simulink model "Board2_supervision"  (R2025b)
settings: Solver=FixedStepDiscrete  StartTime=0.0  StopTime=2  FixedStep=0.001  RelTol=1e-3
(part 2 of 2)

== stateflow chart Board2_supervision/Board2 ==
  state Supervision_task
    state Board_state [parallel]
      settings: executionOrder=1
      state Normal
        ex: Close_Session(); Lower_MTalk(); Abort_Communication();
        state Supervisor [parallel]
          settings: executionOrder=1
          state Waiting_comunication
            en: Update_Local_State(); Open_Session(); Raise_MTalk();
            time_comm = Get_Timestamp();
          state Transmit_Local_State
            en: Send_Local_State(); time_comm = Get_Timestamp();
          state Local_state_transmitted
            en: time_comm = Get_Timestamp();
          state Receive_state
            en: Wait_State(); Lower_MTalk(); time_comm = Get_Timestamp();
          state State_received
            en: Raise_MTalk(); time_comm = Get_Timestamp();
          state Transmit_Global_State
            en: Send_Global_State(); time_comm = Get_Timestamp();
          state Global_Local_state_transmitted
            en: time_comm = Get_Timestamp();
          state Receive_global_state
            en: Wait_Global_State(); Lower_MTalk(); time_comm = Get_Timestamp();
          state Same_decision
            en: Write_Output();
          state Global_state_received
            en: time_comm = Get_Timestamp();
          state Transmit_Decision
            en: Send_Decision(); time_comm = Get_Timestamp();
          state Decision_transmitted
            en: time_comm = Get_Timestamp();
          state Receive_decision
            en: Wait_Decision(); Lower_MTalk(); time_comm = Get_Timestamp();
          (default) -> Waiting_comunication
          (junction 6516) -> Waiting_comunication
          Waiting_comunication -> (junction 6517) [order 2] : [Check_Timeout_Us(time_comm, INITIAL_TIMEOUT)]
          Same_decision -> (junction 6516)
          (junction 6517) -> (junction 6543)
          Waiting_comunication -> Transmit_Local_State [order 1] : [~Is_STalk_High()]
              | {retransmitted = 0;}
          (junction 6556) -> Transmit_Local_State
          Transmit_Local_State -> (junction 6595) [order 2] : [Check_Timeout_Us(time_comm, STATE_SEND_TIMEOUT)]
          (junction 6595) -> (junction 6596)
          (junction 6554) -> (junction 6556) [order 1] : [retransmitted < MAX_RETRANSMIT]{retransmitted = retransmitted + 1;}
          Transmit_Local_State -> Local_state_transmitted [order 1] : [Is_Tx_Finished()]
          (junction 6554) -> (junction 6543) [order 2]
          Local_state_transmitted -> (junction 6554) [order 2] : [Check_Timeout_Us(time_comm, WAIT_TIMEOUT)]
          (junction 6543) -> (junction 6547)
          Local_state_transmitted -> Receive_state [order 1] : [Is_STalk_High()]
          (junction 6567) -> Receive_state
          Receive_state -> (junction 6547) [order 2] : [Check_Timeout_Us(time_comm, STATE_RECEIVE_TIMEOUT)]
          (junction 6566) -> (junction 6567)
          (junction 6547) -> (junction 6544)
          Receive_state -> (junction 6549) [order 1] : [Is_Rx_Finished()]
          (junction 6549) -> (junction 6566) [order 2]
          (junction 6549) -> State_received [order 1] : [Verify_State_Integrity()]
              | {send(STEP,Normal.Global_state_compute);
              | Update_Global_State();}
          State_received -> (junction 6544) [order 2] : [Check_Timeout_Us(time_comm, WAIT_TIMEOUT)]
          (junction 6544) -> (junction 6599)
          State_received -> Transmit_Global_State [order 1] : [~Is_STalk_High()]
          Transmit_Global_State -> (junction 6596) [order 2] : [Check_Timeout_Us(time_comm, GLOBAL_STATE_SEND_TIMEOUT)]
          (junction 6591) -> Transmit_Global_State
          (junction 6596) -> (junction 6602)
          (junction 6590) -> (junction 6591) [order 1] : [retransmitted < MAX_RETRANSMIT]{retransmitted = retransmitted + 1;}
          Transmit_Global_State -> Global_Local_state_transmitted [order 1] : [Is_Tx_Finished()]
          Global_Local_state_transmitted -> (junction 6590) [order 2] : [Check_Timeout_Us(time_comm, WAIT_TIMEOUT)]
          (junction 6590) -> (junction 6599) [order 2]
          (junction 6599) -> (junction 6546)
          Global_Local_state_transmitted -> Receive_global_state [order 1] : [Is_STalk_High()]
          Receive_global_state -> (junction 6546) [order 2] : [Check_Timeout_Us(time_comm, GLOBAL_STATE_RECEIVE_TIMEOUT)]
          (junction 6586) -> Receive_global_state
          (junction 6588) -> (junction 6586)
          (junction 6546) -> (junction 6352)
          Receive_global_state -> (junction 6574) [order 1] : [Is_Rx_Finished()]
          (junction 6574) -> (junction 6588) [order 2]
          (junction 6574) -> (junction 6360) [order 1] : [Verify_Global_Integrity()]
              | { send(STEP, Supervision_task.Board_decision); Raise_MTalk();}
          (junction 6365) -> Same_decision [order 1] : [isequal(decision, receivedDecisionPacket.decision)]
          (junction 6360) -> (junction 6361) [order 2]
          (junction 6367) -> (junction 6361)
          (junction 6360) -> Global_state_received [order 1] : [isequal(global_state, receivedGlobalStatePacket.global_state)]
          Global_state_received -> (junction 6352) [order 2] : [Check_Timeout_Us(time_comm, WAIT_TIMEOUT)]
          (junction 6353) -> (junction 6352)
          Global_state_received -> Transmit_Decision [order 1] : [~Is_STalk_High()]
          (junction 6607) -> Transmit_Decision
          Transmit_Decision -> (junction 6602) [order 2] : [Check_Timeout_Us(time_comm, DECISION_SEND_TIMEOUT)]
          (junction 6602) -> (junction 6629)
          (junction 6606) -> (junction 6607) [order 1] : [retransmitted < MAX_RETRANSMIT]{retransmitted = retransmitted + 1;}
          Transmit_Decision -> Decision_transmitted [order 1] : [Is_Tx_Finished()]
          (junction 6606) -> (junction 6353) [order 2]
          Decision_transmitted -> (junction 6606) [order 2] : [Check_Timeout_Us(time_comm, WAIT_TIMEOUT)]
          (junction 6373) -> (junction 6353)
          Decision_transmitted -> Receive_decision [order 1] : [Is_STalk_High()]
          (junction 6617) -> Receive_decision
          Receive_decision -> (junction 6373) [order 2] : [Check_Timeout_Us(time_comm, DECISION_RECEIVE_TIMEOUT)]
          (junction 6619) -> (junction 6617)
          (junction 6631) -> (junction 6373)
          Receive_decision -> (junction 6613) [order 1] : [Is_Rx_Finished()]
          (junction 6613) -> (junction 6619) [order 2]
          (junction 6613) -> (junction 6369) [order 1] : [Verify_Decision_Integrity()]
              | {Close_Session();}
          (junction 6365) -> (junction 6367) [order 2]
          (junction 6369) -> (junction 6365)
          (junction 6629) -> (junction 6631)
        state Global_state_compute [parallel]
          settings: executionOrder=2
          state Moving_obstacle [parallel]
            settings: executionOrder=1
            state Obstacle_from_left [parallel]
              settings: executionOrder=2
              state Moving_obstacle_from_left
                en: moving_from_left = true;
              state Obstacle_left
                en: time_obs_s1 = Get_Timestamp();
              state Waiting
              (junction 8547) -> (junction 8548)
              (junction 8548) -> (junction 8549)
              Moving_obstacle_from_left -> (junction 8547)
              Obstacle_left -> (junction 8548) [order 2] : [STEP && Check_Timeout_Ms(time_obs_s1, OBS_TIMEOUT)]
              (junction 8549) -> Supervision_task.Board_state.Normal.Global_state_compute.Moving_obstacle.Obstacle_from_left.Waiting
              (default) -> Supervision_task.Board_state.Normal.Global_state_compute.Moving_obstacle.Obstacle_from_left.Waiting
              Obstacle_left -> Moving_obstacle_from_left [order 1] : [STEP && Obs_Sonar2()]
              Supervision_task.Board_state.Normal.Global_state_compute.Moving_obstacle.Obstacle_from_left.Waiting -> Obstacle_left : [STEP && Obs_Sonar1() && ~Obs_Sonar2()]
            state Obstacle_from_right [parallel]
              settings: executionOrder=3
              state Waiting
              state Obstacle_right
                en: time_obs_s3 = Get_Timestamp();
              state Moving_obstacle_from_right
                en: moving_from_right = true;
              (junction 8563) -> (junction 8562)
              (junction 8564) -> (junction 8563)
              (junction 8562) -> Supervision_task.Board_state.Normal.Global_state_compute.Moving_obstacle.Obstacle_from_right.Waiting
              Obstacle_right -> (junction 8563) [order 2] : [STEP && Check_Timeout_Ms(time_obs_s3, OBS_TIMEOUT)]
              Moving_obstacle_from_right -> (junction 8564)
              (default) -> Supervision_task.Board_state.Normal.Global_state_compute.Moving_obstacle.Obstacle_from_right.Waiting
              Obstacle_right -> Moving_obstacle_from_right [order 1] : [STEP && Obs_Sonar2()]
              Supervision_task.Board_state.Normal.Global_state_compute.Moving_obstacle.Obstacle_from_right.Waiting -> Obstacle_right : [STEP && Obs_Sonar3() && ~Obs_Sonar2()]
            state No_obstacle [parallel]
              settings: executionOrder=1
              state No_movements
                en: moving_from_left = false;
                moving_from_right = false;
              (default) -> No_movements
              No_movements -> No_movements : [STEP]
          state Battery_temperature_manager [parallel]
            settings: executionOrder=2
            state Temperature_manager [parallel]
              settings: executionOrder=3
              state High_temperature
                en: time_temp = Get_Timestamp();
              state Normal
              state Limited
                en: limit_velocity = true;
              High_temperature -> (junction 8657) [order 1] : [STEP && Check_Timeout_Ms(time_temp, TEMP_TIMEOUT)]
              (junction 8656) -> High_temperature
              (junction 8657) -> Supervision_task.Board_state.Normal.Global_state_compute.Battery_temperature_manager.Temperature_manager.Limited
              Supervision_task.Board_state.Normal.Global_state_compute.Battery_temperature_manager.Temperature_manager.Normal -> (junction 8656) : [STEP && High_Temp()]
              High_temperature -> (junction 8658) [order 2] : [STEP && ~High_Temp()]
              (default) -> Supervision_task.Board_state.Normal.Global_state_compute.Battery_temperature_manager.Temperature_manager.Normal
              (junction 8658) -> Supervision_task.Board_state.Normal.Global_state_compute.Battery_temperature_manager.Temperature_manager.Normal
              Supervision_task.Board_state.Normal.Global_state_compute.Battery_temperature_manager.Temperature_manager.Limited -> (junction 8658) [order 1] : [STEP && ~High_Temp()]
              Supervision_task.Board_state.Normal.Global_state_compute.Battery_temperature_manager.Temperature_manager.Limited -> Supervision_task.Board_state.Normal.Global_state_compute.Battery_temperature_manager.Temperature_manager.Limited [order 2] : [STEP]
            state Battery_manager [parallel]
              settings: executionOrder=2
              state Normal
              state Limited
                en: limit_velocity = true;
              Supervision_task.Board_state.Normal.Global_state_compute.Battery_temperature_manager.Battery_manager.Limited -> Supervision_task.Board_state.Normal.Global_state_compute.Battery_temperature_manager.Battery_manager.Limited [order 2] : [STEP]
              (default) -> Supervision_task.Board_state.Normal.Global_state_compute.Battery_temperature_manager.Battery_manager.Normal
              Supervision_task.Board_state.Normal.Global_state_compute.Battery_temperature_manager.Battery_manager.Normal -> Supervision_task.Board_state.Normal.Global_state_compute.Battery_temperature_manager.Battery_manager.Limited : [STEP && Low_Voltage()]
              (junction 8674) -> Supervision_task.Board_state.Normal.Global_state_compute.Battery_temperature_manager.Battery_manager.Normal
              Supervision_task.Board_state.Normal.Global_state_compute.Battery_temperature_manager.Battery_manager.Limited -> (junction 8675) [order 1]
              (junction 8675) -> (junction 8674) : [STEP && ~Low_Voltage()]
            state Normal_velocity [parallel]
              settings: executionOrder=1
              state No_limitation
                en: limit_velocity = false;
              (default) -> No_limitation
              No_limitation -> No_limitation : [STEP]
          state Combo [parallel]
            settings: executionOrder=3
            state Special_retro_change
              en: special_retro = ~special_retro;
            state Obs_detection_change
              en: obs_detection = ~obs_detection;
            state Button1_pressed_combo
              en: time_button = Get_Timestamp();
            state Waiting_combo
            state Button2_pressed_combo
              en: time_button = Get_Timestamp();
            state Max_velocity_decrease
              en: change_velocity = - int8(VEL_CHANGE);
            state Max_velocity_increase
              en: change_velocity = int8(VEL_CHANGE);
            Special_retro_change -> (junction 11480)
            Obs_detection_change -> (junction 11480)
            (junction 11480) -> Waiting_combo
            Button1_pressed_combo -> Special_retro_change [order 1] : [Button2_Pressed()]
            Button2_pressed_combo -> Obs_detection_change [order 1] : [Button1_Pressed()]
            (default) -> Waiting_combo
            Waiting_combo -> Button2_pressed_combo [order 2] : [Button2_Pressed()]
            Waiting_combo -> Button1_pressed_combo [order 1] : [Button1_Pressed()]
            Button1_pressed_combo -> Waiting_combo [order 3] : [STEP && Check_Timeout_Ms(time_button, BUTTON_TIMEOUT)]
            Button2_pressed_combo -> Waiting_combo [order 3] : [STEP && Check_Timeout_Ms(time_button, BUTTON_TIMEOUT)]
            Button1_pressed_combo -> Max_velocity_decrease [order 2] : [Button1_Pressed()]
            (junction 11489) -> Waiting_combo
            Button2_pressed_combo -> Max_velocity_increase [order 2] : [Button2_Pressed()]
            Max_velocity_decrease -> (junction 11489)
            Max_velocity_increase -> (junction 11489)
      state Single_Board
        state Other_board_failure
          en: Compute_Degraded_Actions();
        Other_board_failure -> Other_board_failure
        (default) -> Other_board_failure
      state Degraded
        state Restablish
          state Starting_to_restablish
            en: Open_Session(); Raise_MTalk(); time_comm = Get_Timestamp();
          state Transmit_ping
            en: Send_Ping(); time_comm = Get_Timestamp();
          state Ping_transmitted
            en: time_comm = Get_Timestamp();
          state Receive_ping
            en: Wait_Ping(); Lower_MTalk(); time_comm = Get_Timestamp();
          state Connection_restablished
          (junction 3631) -> (junction 3889)
          (junction 5962) -> (junction 3631)
          (junction 3889) -> (junction 3901)
          (default) -> Starting_to_restablish : {Compute_Degraded_Actions();}
          Starting_to_restablish -> (junction 3901) [order 2] : [Check_Timeout_Us(time_comm, INITIAL_TIMEOUT)]
          (junction 3901) -> (junction 3170)
          Starting_to_restablish -> Transmit_ping [order 1] : [~Is_STalk_High()]
              | {retransmitted = 0;}
          (junction 6638) -> Transmit_ping
          Transmit_ping -> (junction 5962) [order 2] : [Check_Timeout_Us(time_comm, BYTE_SEND_TIMEOUT)]
          (junction 6639) -> (junction 6638) [order 1] : [retransmitted < MAX_RETRANSMIT]{retransmitted = retransmitted + 1;}
          (junction 6659) -> (junction 3170)
          Transmit_ping -> Ping_transmitted [order 1] : [Is_Tx_Finished()]
          Ping_transmitted -> (junction 6639) [order 2] : [Check_Timeout_Us(time_comm, WAIT_TIMEOUT)]
          (junction 6639) -> (junction 6659) [order 2]
          (junction 3181) -> (junction 6659)
          Ping_transmitted -> Receive_ping [order 1] : [Is_STalk_High()]
          (junction 6655) -> Receive_ping
          Receive_ping -> (junction 3181) [order 2] : [Check_Timeout_Us(time_comm, BYTE_RECEIVE_TIMEOUT)]
          (junction 6657) -> (junction 6655)
          Receive_ping -> (junction 6640) [order 1] : [Is_Rx_Finished()]
          (junction 6640) -> (junction 6657) [order 2]
          (junction 6640) -> Connection_restablished [order 1] : [Verify_Ping()]
              | {Close_Session();}
        state Restarting
        (default) -> Restarting
        Restarting -> Restablish
        (junction 3170) -> Restarting : {Abort_Communication(); Close_Session(); Lower_MTalk();}
      (default) -> Supervision_task.Board_state.Normal
      (junction 6352) -> Degraded : {Compute_Degraded_Actions();}
      (junction 6361) -> Single_Board
      Connection_restablished -> Supervision_task.Board_state.Normal
    state Board_decision [parallel]
      settings: executionOrder=2
      state Working_status_manager [parallel]
        settings: executionOrder=1
        state Init_working
        state Motor_error_working
          en: working_status = ...
          WORKING_STATUS_TYPE.MOTOR_ERROR_WORKING;
        state Normal_working
          en: working_status = ...
          WORKING_STATUS_TYPE.NORMAL_WORKING;
        state Critical_voltage_working
          en: working_status = ...
          WORKING_STATUS_TYPE.CRITICAL_VOLTAGE_WORKING;
        (default) -> Init_working : {init_count = 0;}
        (junction 13208) -> Init_working
        (junction 13206) -> (junction 13208)
        Init_working -> (junction 13203) : [STEP]{init_count = init_count + 1;}
        (junction 13203) -> (junction 13206) [order 2]
        (junction 13203) -> (junction 13211) [order 1] : [init_count >= INIT_COUNTER]
        (junction 13211) -> (junction 13218) [order 1] : [Motor_Error()]
        (junction 13211) -> (junction 13221) [order 2] : [Critical_Voltage()]
        (junction 13218) -> Motor_error_working
        (junction 13211) -> Normal_working [order 3]
        (junction 13221) -> Critical_voltage_working
        Normal_working -> Critical_voltage_working [order 2] : [STEP && Critical_Voltage()]
        Normal_working -> Motor_error_working [order 1] : [STEP && Motor_Error()]
        Critical_voltage_working -> Normal_working : [~Critical_Voltage()]
      state Routine_manager [parallel]
        settings: executionOrder=4
        state Max_velocity_handler [parallel]
          settings: executionOrder=1
          state Waiting_change_max_vel
          Waiting_change_max_vel -> Waiting_change_max_vel [order 1] : [Detect_Limit_Activation()]
          (default) -> Waiting_change_max_vel
          Waiting_change_max_vel -> (junction 12774) [order 3] : [STEP && global_state.change_vel == - int8(VEL_CHANGE)]
              | {Decrease_Max_Vel();}
          Waiting_change_max_vel -> (junction 12775) [order 2] : [STEP && global_state.change_vel == int8(VEL_CHANGE)]
              | {Increase_Max_Vel();}
          (junction 12774) -> (junction 12776)
          (junction 12775) -> (junction 12778)
          (junction 12777) -> Waiting_change_max_vel
          (junction 12776) -> (junction 12777)
          (junction 12778) -> (junction 12777)
        state Compute_routine [parallel]
          settings: executionOrder=2
          state Routine_state_normal
            state Motor_error_routine
              en: Stop_Motors();
              decision.brk_mode = BRAKING_TYPE.EMERGENCY;
            state Critical_voltage_routine
              en: Stop_Motors();
              decision.brk_mode = BRAKING_TYPE.EMERGENCY;
            state Normal_routine
              state Low_controller_battery_routine
                state Control_battery_stop
                  en: Stop_Motors();
                  decision.brk_mode = BRAKING_TYPE.NORMAL;
                (default) -> Control_battery_stop
              state Special_retro_routine
                ex: special_retro_rotating = false;
                state Turn_back_gyro
                  en: Turn_Back(); decision.brk_mode = BRAKING_TYPE.NONE;
                state Turn_back_no_gyro
                  en: Turn_Back(); decision.brk_mode = BRAKING_TYPE.NONE;
                state Stop_back_rotation
                  en: Stop_Motors(); decision.brk_mode = BRAKING_TYPE.NONE;
                (default) -> (junction 13723) : {special_retro_rotating = true; turn_counter = 0;}
                (junction 13723) -> Turn_back_no_gyro [order 2]
                (junction 13722) -> Turn_back_gyro
                (junction 13723) -> Turn_back_gyro [order 1] : [~global_state.stateB2.gyroError]
                    | {angle = 0; prevYaw = 0;}
                (junction 13724) -> Turn_back_no_gyro
                (junction 13725) -> (junction 13722)
                (junction 13729) -> (junction 13724)
                Turn_back_gyro -> (junction 13726) : [STEP]{Update_Angle(global_state.stateB2.gyroYaw);
                    | turn_counter = turn_counter + 1;}
                Turn_back_no_gyro -> (junction 13728) : [STEP]{turn_counter = turn_counter + 1;}
                (junction 13726) -> (junction 13727) [order 1] : [abs(angle) >= TURN_BACK_ANGLE || turn_counter >= TURN_BACK_LIMIT_COUNT]
                    | {angle = 0; prevYaw = 0;}
                (junction 13728) -> (junction 13727) [order 1] : [turn_counter >= TURN_BACK_COUNT]
                (junction 13726) -> (junction 13725) [order 2]
                (junction 13728) -> (junction 13729) [order 2]
                (junction 13727) -> Stop_back_rotation : {turn_counter = 0;}
                Stop_back_rotation -> (junction 13730) : [global_state.stateB2.controller_y >= CONTROLLER_ZERO]
                (junction 13730) -> (junction 13731)
              state Emergency_button_routine
                state Emergency_button
                  en: Stop_Motors();
                  decision.brk_mode = BRAKING_TYPE.EMERGENCY;
                (default) -> Emergency_button
                Emergency_button -> (junction 13551) : [Is_Rover_Stationary()]
                (junction 13551) -> (junction 13552)
              state Stop_slow_routine
                state Stop_slow
                  en: Stop_Motors();
                  decision.brk_mode = BRAKING_TYPE.NORMAL;
                (default) -> Stop_slow
                Stop_slow -> (junction 13713) : [Is_Rover_Stationary()]
                (junction 13713) -> (junction 13714)
              state Moving_obstacle_from_left_routine
                state Turn_moving_left_no_gyro
                  en: Process_Evasive_Commands(false, open_loop);
                  decision.brk_mode = BRAKING_TYPE.NONE;
                state Turn_moving_left_gyro
                  en: Process_Evasive_Commands(false, open_loop);
                  decision.brk_mode = BRAKING_TYPE.NONE;
                (default) -> (junction 13647) : {turn_counter = 0;}
                (junction 13646) -> Turn_moving_left_no_gyro
                (junction 13647) -> Turn_moving_left_gyro [order 1] : [~global_state.stateB2.gyroError]
                    | {angle = 0; prevYaw = 0;}
                (junction 13648) -> Turn_moving_left_gyro
                (junction 13647) -> Turn_moving_left_no_gyro [order 2]
                (junction 13649) -> (junction 13646)
                (junction 13653) -> (junction 13648)
                Turn_moving_left_gyro -> (junction 13652) : [STEP]{Update_Angle(global_state.stateB2.gyroYaw);
                    | turn_counter = turn_counter + 1;}
                Turn_moving_left_no_gyro -> (junction 13650) : [STEP]{turn_counter = turn_counter + 1;}
                (junction 13650) -> (junction 13649) [order 2]
                (junction 13650) -> (junction 13651) [order 1] : [turn_counter >= TURN_COUNT]
                (junction 13652) -> (junction 13651) [order 1] : [abs(angle) >= TURN_ANGLE || turn_counter >= TURN_LIMIT_COUNT]
                    | {angle = 0; prevYaw = 0;}
                (junction 13652) -> (junction 13653) [order 2]
                (junction 13651) -> (junction 13654) : {turn_counter = 0;}
                (junction 13654) -> (junction 13655)
              state Emergency_sonar_routine
                state Emergency_sonar
                  en: Stop_Motors();
                  decision.brk_mode = BRAKING_TYPE.EMERGENCY;
                state Turn_left_no_gyro
                  en: Turn_Left(); decision.brk_mode = BRAKING_TYPE.NONE;
                state Turn_right_no_gyro
                  en: Turn_Right(); decision.brk_mode = BRAKING_TYPE.NONE;
                state Turn_right_gyro
                  en: Turn_Right(); decision.brk_mode = BRAKING_TYPE.NONE;
                state Turn_left
                  en: Turn_Left(); decision.brk_mode = BRAKING_TYPE.NONE;
                state Stop_left_rotation
                  en: Stop_Motors(); decision.brk_mode = BRAKING_TYPE.NONE;
                state Stop_right_rotation
                  en: Stop_Motors(); decision.brk_mode = BRAKING_TYPE.NONE;
                (default) -> Emergency_sonar
                Emergency_sonar -> (junction 13566) : [STEP && Is_Rover_Stationary()]
                (junction 13566) -> (junction 13565) [order 2] : [global_state.stateB2.sonar1 > distance_threshold]
                (junction 13566) -> (junction 13567) [order 1] : [global_state.stateB2.sonar3 > distance_threshold]
                (junction 13566) -> (junction 13588) [order 3]
                (junction 13565) -> (junction 13569) : {turn_counter = 0;}
                (junction 13567) -> (junction 13572) : {turn_counter = 0;}
                (junction 13569) -> (junction 13570) [order 2]
                (junction 13572) -> (junction 13571) [order 2]
                (junction 13569) -> (junction 13568) [order 1] : [~global_state.stateB2.gyroError]
                    | {angle = 0; prevYaw = 0;}
                (junction 13572) -> (junction 13573) [order 1] : [~global_state.stateB2.gyroError]
                    | {angle = 0; prevYaw = 0;}
                (junction 13568) -> Turn_left
                (junction 13570) -> Turn_left_no_gyro
                (junction 13571) -> Turn_right_no_gyro
                (junction 13573) -> Turn_right_gyro
                (junction 13574) -> Turn_left_no_gyro
                (junction 13575) -> Turn_right_no_gyro
                (junction 13576) -> Turn_right_gyro
                (junction 13582) -> (junction 13574)
                (junction 13583) -> (junction 13575)
                (junction 13587) -> (junction 13576)
                (junction 13577) -> Turn_left
                (junction 13578) -> (junction 13577)
                Turn_right_gyro -> (junction 13586) : [STEP]{Update_Angle(global_state.stateB2.gyroYaw);
                    | turn_counter = turn_counter + 1;}
                Turn_left_no_gyro -> (junction 13581) : [STEP]{turn_counter = turn_counter + 1;}
                Turn_right_no_gyro -> (junction 13584) : [STEP]{turn_counter = turn_counter + 1;}
                Turn_left -> (junction 13579) : [STEP]{Update_Angle(global_state.stateB2.gyroYaw);
                    | turn_counter = turn_counter + 1;}
                (junction 13579) -> (junction 13580) [order 1] : [abs(angle) >= TURN_ANGLE || turn_counter >= TURN_LIMIT_COUNT]
                    | {angle = 0; prevYaw = 0;}
                (junction 13581) -> (junction 13580) [order 1] : [turn_counter >= TURN_COUNT]
                (junction 13584) -> (junction 13585) [order 1] : [turn_counter >= TURN_COUNT]
                (junction 13586) -> (junction 13585) [order 1] : [abs(angle) >= TURN_ANGLE || turn_counter >= TURN_LIMIT_COUNT]
                    | {angle = 0; prevYaw = 0;}
                (junction 13579) -> (junction 13578) [order 2]
                (junction 13581) -> (junction 13582) [order 2]
                (junction 13584) -> (junction 13583) [order 2]
                (junction 13586) -> (junction 13587) [order 2]
                (junction 13580) -> Stop_left_rotation : {turn_counter = 0;}
                (junction 13585) -> Stop_right_rotation : {turn_counter = 0;}
                Stop_left_rotation -> (junction 13588)
                Stop_right_rotation -> (junction 13588)
                (junction 13588) -> (junction 13589)
                (junction 13589) -> (junction 13590)
              state Moving_obstacle_from_right_routine
                state Turn_moving_right_no_gyro
                  en: Process_Evasive_Commands(true, open_loop);
                  decision.brk_mode = BRAKING_TYPE.NONE;
                state Turn_moving_right_gyro
                  en: Process_Evasive_Commands(true, open_loop);
                  decision.brk_mode = BRAKING_TYPE.NONE;
                (default) -> (junction 13680) : {turn_counter = 0;}
                (junction 13679) -> Turn_moving_right_no_gyro
                (junction 13680) -> Turn_moving_right_gyro [order 1] : [~global_state.stateB2.gyroError]
                    | {angle = 0; prevYaw = 0;}
                (junction 13680) -> Turn_moving_right_no_gyro [order 2]
                (junction 13681) -> Turn_moving_right_gyro
                (junction 13682) -> (junction 13679)
                (junction 13686) -> (junction 13681)
                Turn_moving_right_gyro -> (junction 13685) : [STEP]{Update_Angle(global_state.stateB2.gyroYaw);
                    | turn_counter = turn_counter + 1;}
                Turn_moving_right_no_gyro -> (junction 13683) : [STEP]{turn_counter = turn_counter + 1;}
                (junction 13683) -> (junction 13682) [order 2]
                (junction 13685) -> (junction 13686) [order 2]
                (junction 13683) -> (junction 13684) [order 1] : [turn_counter >= TURN_COUNT]
                (junction 13685) -> (junction 13684) [order 1] : [abs(angle) >= TURN_ANGLE || turn_counter >= TURN_LIMIT_COUNT]
                    | {angle = 0; prevYaw = 0;}
                (junction 13684) -> (junction 13687) : {turn_counter = 0;}
                (junction 13687) -> (junction 13688)
              state Select_routine
              state Control_controller_routine
                state Control_from_controller
                  en: Process_User_Commands(open_loop); decision.brk_mode = BRAKING_TYPE.NONE;
                (default) -> Control_from_controller
              state Not_moving_routine
                state Not_moving
                  en: Stop_Motors();
                  decision.brk_mode = BRAKING_TYPE.NORMAL;
                (default) -> Not_moving
              (junction 13655) -> Select_routine
              (junction 13532) -> (junction 13531)
              (junction 13545) -> (junction 13532)
              (junction 13546) -> (junction 13545)
              (junction 13528) -> (junction 13546)
              (junction 13531) -> Emergency_button_routine
              Moving_obstacle_from_right_routine -> (junction 13532) [order 1] : [Emergency_B_Pressed()]
              Moving_obstacle_from_left_routine -> (junction 13545) [order 1] : [Emergency_B_Pressed()]
              Stop_slow_routine -> (junction 13546) [order 1] : [Emergency_B_Pressed()]
              Special_retro_routine -> (junction 13528) [order 1] : [Emergency_B_Pressed()]
              (junction 13552) -> Select_routine
              (junction 13534) -> (junction 13533)
              (junction 13547) -> (junction 13534)
              (junction 13548) -> (junction 13547)
              (junction 13533) -> Emergency_sonar_routine
              Moving_obstacle_from_right_routine -> (junction 13534) [order 2] : [Near_Obstacle()]
              Moving_obstacle_from_left_routine -> (junction 13547) [order 2] : [Near_Obstacle()]
              Stop_slow_routine -> (junction 13548) [order 2] : [Near_Obstacle()]
              (junction 13815) -> (junction 13549)
              (junction 13549) -> Moving_obstacle_from_right_routine
              Stop_slow_routine -> (junction 13815) [order 3] : [Mov_Obs_Right()]
              (junction 13819) -> (junction 13816)
              (junction 13816) -> (junction 13814)
              (junction 13826) -> (junction 13814)
              Moving_obstacle_from_right_routine -> (junction 13819) [order 3] : [Stop_B_Pressed()]
              Moving_obstacle_from_left_routine -> (junction 13816) [order 3] : [Stop_B_Pressed()]
              (junction 13814) -> Stop_slow_routine
              Special_retro_routine -> (junction 13826) [order 2] : [Stop_B_Pressed()]
              Not_moving -> Select_routine
              Control_from_controller -> Select_routine
              (junction 13714) -> Select_routine
              (junction 13731) -> Select_routine
              Control_battery_stop -> Select_routine
              Stop_slow_routine -> Moving_obstacle_from_left_routine [order 4] : [Mov_Obs_Left()]
              (junction 13688) -> Select_routine
              Emergency_sonar_routine -> Emergency_button_routine : [Emergency_B_Pressed()]
              Select_routine -> Emergency_button_routine [order 1] : [Emergency_B_Routine()]
              Select_routine -> Emergency_sonar_routine [order 2] : [Emergency_S_Routine()]
              Select_routine -> Moving_obstacle_from_right_routine [order 3] : [Mov_Obs_R_Routine()]
              Select_routine -> Moving_obstacle_from_left_routine [order 4] : [Mov_Obs_L_Routine()]
              Select_routine -> Stop_slow_routine [order 5] : [Stop_Slow_Routine()]
              Select_routine -> Low_controller_battery_routine [order 6] : [Low_Controller_Battery_Routine()]
              Select_routine -> Special_retro_routine [order 7] : [Spec_Retro_Routine()]
              (default) -> Select_routine
              (junction 13590) -> Select_routine
              Select_routine -> Control_controller_routine [order 9] : [STEP]
              Select_routine -> Not_moving_routine [order 8] : [Stationary_Obs_Routine()]
            Normal_routine -> Motor_error_routine [order 1] : [STEP && Motor_Error_Occured()]
            Critical_voltage_routine -> Normal_routine : [~Critical_Voltage_Occured()]
            Normal_routine -> Critical_voltage_routine [order 2] : [STEP && Critical_Voltage_Occured()]
            (default) -> Normal_routine
          (default) -> Routine_state_normal
          Routine_state_normal -> Routine_state_normal : [in(Board_state.Degraded)]
      state Mode_manager [parallel]
        settings: executionOrder=5
        state Normal_driving
          state Mode_DEFAULT
            en: decision.mode = ...
            ROVER_MODE.DEFAULT;
          state Mode_SPORT
            en: decision.mode = ...
            ROVER_MODE.SPORT;
          state Mode_ECO
            en: decision.mode = ...
            ROVER_MODE.ECO;
          (default) -> Mode_DEFAULT
          Mode_SPORT -> Mode_ECO : [Mode_B_Pressed()]
          Mode_DEFAULT -> Mode_SPORT : [Mode_B_Pressed()]
          (junction 13114) -> Mode_DEFAULT
          Mode_ECO -> (junction 13115) : [Mode_B_Pressed()]
          (junction 13115) -> (junction 13114)
        state Critical_voltage_driving
          en: decision.mode = ...
          ROVER_MODE.ECO;
        state Motor_error_driving
          en: decision.mode = ...
          ROVER_MODE.DEFAULT;
        (default) -> Normal_driving
        Normal_driving -> Critical_voltage_driving [order 2] : [STEP && Critical_Voltage_Occured()]
        Critical_voltage_driving -> Normal_driving : [~Critical_Voltage_Occured()]
        Normal_driving -> Motor_error_driving [order 1] : [STEP && Motor_Error_Occured()]
      state Relay_manager [parallel]
        settings: executionOrder=2
        state Motor_error_relay
          en: decision.relay = false;
        state Normal_relay
          en: decision.relay = true;
        state Critical_voltage_relay
          en: decision.relay = false;
        (default) -> Normal_relay
        Normal_relay -> Motor_error_relay [order 1] : [STEP && Motor_Error_Occured()]
        Normal_relay -> Critical_voltage_relay [order 2] : [STEP && Critical_Voltage_Occured()]
        (junction 13149) -> Normal_relay
        Critical_voltage_relay -> (junction 13150) : [~Critical_Voltage_Occured()]
        (junction 13150) -> (junction 13149)
      state Lights_manager [parallel]
        settings: executionOrder=6
        state Normal_lights
          state Lights_OFF
            en: Rover_Lights_OFF();
          state Lights_ON
            en: Update_Rover_Lights(true);
          state Lights_AUTO
            en: Update_Rover_Lights(false);
          Lights_ON -> Lights_ON [order 2] : [STEP]
          Lights_AUTO -> Lights_AUTO [order 2] : [STEP]
          (default) -> Lights_OFF
          Lights_ON -> Lights_AUTO [order 1] : [Lights_B_Pressed()]
          Lights_OFF -> Lights_ON : [Lights_B_Pressed()]
          (junction 13168) -> Lights_OFF
          Lights_AUTO -> (junction 13169) [order 1] : [Lights_B_Pressed()]
          (junction 13169) -> (junction 13168)
        state Critical_voltage_lights
          en: Rover_Lights_OFF();
        state Motor_error_lights
          en: Rover_Lights_Motor_Error();
        (default) -> Normal_lights
        Normal_lights -> Critical_voltage_lights [order 2] : [STEP && Critical_Voltage_Occured()]
        Critical_voltage_lights -> Normal_lights : [~Critical_Voltage_Occured()]
        Normal_lights -> Motor_error_lights [order 1] : [STEP && Motor_Error_Occured()]
      state Mux_manager [parallel]
        settings: executionOrder=3
        state Normal_mux
          en: decision.mux = false;
        state Degraded_mux
          en: decision.mux = true; open_loop = true;
          ex: open_loop = false;
        (default) -> Normal_mux
        Normal_mux -> Degraded_mux : [in(Board_state.Degraded)]
        (junction 13188) -> Normal_mux
        Degraded_mux -> (junction 13189) : [STEP && in(Board_state.Normal) && Is_Rover_Stationary()]
        (junction 13189) -> (junction 13188)
  (default) -> Supervision_task : {Init_Data(); Lower_MTalk();}
  data: y function_output; y function_output; y function_output; y function_output; y function_output; y function_output; y function_output; y function_output; y function_output; y function_output; y function_output; y function_output; start_time function_input; min_elapsed_time function_input; y function_output; start_time function_input; min_elapsed_time function_input; y function_output; y function_output; y function_output; y function_output; y function_output; y function_output; y function_output; turn_right function_input; opn_loop function_input; opn_loop function_input; yaw function_input; y function_output; y function_output; y function_output; y function_output; y function_output; y function_output; y function_output; y function_output; y function_output; y function_output; y function_output; y function_output; y function_output; y function_output; y function_output; y function_output; y function_output; y function_output; white_led_when_stopped function_input; y function_output; sonar1 input uint16; sonar2 input uint16; sonar3 input uint16; controller_x input uint16; controller_y input uint16; retransmitted local uint8; state local Bus: StateBusB2; global_state local Bus: GSBus; decision local Bus: DecBus; OBS_TIMEOUT constant uint32 =1000; MIN_DISTANCE constant uint16 =150; MAX_DISTANCE constant uint16 =300; B1 input boolean; B2 input boolean; IMM_DISTANCE constant uint16 =70; BUTTON_TIMEOUT constant uint32 =700; special_retro local boolean; gyroYaw input single; LOW_VOLTAGE constant single =9.83; HIGH_TEMPERATURE constant single =100; angle local single; limit_velocity local boolean =false; receivedStatePacket local Bus: PacketStateB1; receivedDecisionPacket local Bus: PacketDecision; receivedGlobalStatePacket local Bus: PacketGstate; receivedPing local uint8 =0; output output Bus: DecBus; MAX_RPM constant uint8 =150; LIMITED_RPM constant uint8 =80; TURN_RPM constant single =20; prevYaw local single; PERIOD constant single =0.06; TEMP_TIMEOUT constant uint32 =10000; time_temp local uint32; time_obs_s1 local uint32; CONTROLLER_ZERO constant uint16 =255; PURE_TURN_EPS constant single =0.01; TURN_RATIO constant single =0.35; CENTER constant single =255; time_comm local uint32; TURN_THRESHOLD local single =5; TURN_ANGLE constant single =45; TURN_BACK_ANGLE constant single =180; B3 input boolean; B4 input boolean; B_r_stick input boolean; controller_battery input uint8; CRITICAL_VOLTAGE constant single =9; LOW_CONTROLLER_BATTERY constant uint8 =5; TURN_BACK_RPM constant single =40; BYTE_RECEIVE_TIMEOUT constant uint32 =1000; BYTE_SEND_TIMEOUT constant uint32 =500; DECISION_RECEIVE_TIMEOUT constant uint32 =3500; DECISION_SEND_TIMEOUT constant uint32 =3000; GLOBAL_STATE_RECEIVE_TIMEOUT constant uint32 =5900; INITIAL_TIMEOUT constant uint32 =1500; STATE_RECEIVE_TIMEOUT constant uint32 =3100; STATE_SEND_TIMEOUT constant uint32 =3000; GLOBAL_STATE_SEND_TIMEOUT constant uint32 =5400; WAIT_TIMEOUT constant uint32 =500; MAX_RETRANSMIT constant uint8 =1; B_l_stick input boolean; obs_detection local boolean; PROTECTION_DISTANCE constant uint16 =40; distance_threshold local uint16 =0; STOP_THRESHOLD constant uint16 =1; time_obs_s3 local uint32; max_velocity local uint8; VEL_CHANGE constant uint8 =10; MIN_RPM constant uint8 =50; MIN_TURN_SCALE_EVASIVE constant single =0.2; MAX_TURN_SCALE_EVASIVE constant single =0.5; special_retro_rotating local boolean =false; change_velocity local int8 =0; moving_from_left local boolean =false; moving_from_right local boolean =false; controllerError input boolean; gyroError input boolean; turn_counter local uint8; TURN_BACK_COUNT constant uint32 =40; TURN_COUNT constant uint8 =20; working_status local Enum: WORKING_STATUS_TYPE =WORKING_STATUS_TYPE.NORMAL_WORKING; time_button local uint32; open_loop local boolean =false; panic_lockdown local boolean =false; init_count local uint8; INIT_COUNTER constant uint8 =35; TURN_BACK_LIMIT_COUNT constant uint8 =50; TURN_LIMIT_COUNT constant uint8 =30
  events: STEP local FUNCTION_CALL_EVENT
  function Lower_MTalk:
    | function Lower_MTalk
    | % Porta a livello basso logico (0) la linea di controllo Master Talk (M_TALK).
    | %
    | % Descrizione:
    | %   Questa funzione agisce sull'hardware della Board 2 (Master). 
    | %   Nel protocollo di handshake asincrono, l'abbassamento di M_TALK viene usato per:
    | %   1. Resettare la linea in fase di inizializzazione o gestione errori.
    | %   2. Cedere il controllo del bus allo Slave (Board 1) dopo che il Master 
    | %      ha ricevuto l'ACK (S_TALK = 1) dallo Slave.
    | %   3. Predisporsi alla ricezione del pacchetto di risposta dello Slave.
    | % 
    | % Dipendenze:
    | %   Richiede 'board2_functions.h' e l'implementazione C di 'reIO_Set_MasterTalk'.
    | 
    |     coder.cinclude('board2_functions.h');
    |     coder.ceval('IO_Reset_MasterTalk');
    | end
  function Init_Data:
    | function Init_Data
    | % Inizializzazione globale del sistema e configurazione di default.
    | %
    | % Descrizione:
    | %   Questa funzione prepara l'ambiente di lavoro iniziale:
    | %   1. Richiama i costruttori per tutte le strutture dati complesse
    | %   2. Imposta le variabili operative di default.
    | 
    |     % Inizializzazione stati logici
    |     state = Init_State(); 
    |     global_state = Init_Global_State(); 
    |     decision = Init_Decision();
    |     
    |     % Inizializzazione pacchetti di comunicazione (payload + CRC)
    |     receivedStatePacket = Init_State_Packet(); 
    |     receivedGlobalStatePacket = Init_Global_State_Packet(); 
    |     receivedDecisionPacket = Init_Decision_Packet();
    | 
    |      % Inizializzazione variabili operative
    |     special_retro = true;
    |     obs_detection= true;
    |     max_velocity = MAX_RPM;
    |     
    | end
    | 
    | 
    | function y = Init_State()
    | % Inizializza la struttura dei dati provenienti dai sensori.
    | %
    | % Descrizione:
    | %   Contiene i dati grezzi acquisiti dalla scheda: IMU (accelerometro/giroscopio),
    | %   sensori di distanza (sonar) e stato del controller (joystick/pulsanti).
    | %
    | % Output:
    | %   - y: Struct contenente i campi sensori inizializzati a 0 o false.
    | 
    |     y.gyroYaw = single(0);        % Velocità angolare Yaw (rad/s o deg/s)
    |     
    |     y.sonar1 = uint16(0);         % Distanza Sonar 1
    |     y.sonar2 = uint16(0);         % Distanza Sonar 2
    |     y.sonar3 = uint16(0);         % Distanza Sonar 3
    |     
    |     y.controller_y = uint16(0);   % Input asse Y Joystick
    |     y.controller_x = uint16(0);   % Input asse X Joystick
    |     
    |     % Stato pulsanti controller (Boolean)
    |     y.button1 = false;
    |     y.button2 = false;
    |     y.button3 = false;
    |     y.button4 = false;
    |     y.r_stick_button = false;
    |     y.l_stick_button = false;
    |     
    |     y.controller_battery = uint8(0); % Livello batteria controller
    | 
    |     y.controllerError = false;
    |     y.gyroError = false;
    | end
    | 
    | function y = initRecState
    | % Inizializza la struttura dei dati provenienti dai sensori dell'altra
    | % board.
    | %
    | % Descrizione:
    | %   Contiene i dati grezzi acquisiti dalla scheda: batteria,
    | %   sensore di temperatura interno e velocità dei motori.
    | %
    | % Output:
    | %   - y: Struct contenente i campi sensori inizializzati a 0.
    | 
    |     y.battery_voltage = single(0); % Tensione batteria principale
    |     y.temperature = single(0);     % Temperatura sistema/driver
    |     
    |     % Velocità lette dagli encoder (Front/Back - A/B)
    |     y.velocity_FA = int16(0);
    |     y.velocity_FB = int16(0);
    |     y.velocity_BA = int16(0);
    |     y.velocity_BB = int16(0);
    |     y.motorError_FA = false;
    |     y.motorError_FB = false;
    |     y.motorError_BA = false;
    |     y.motorError_BB = false;
    | 
    | end
    | 
    | 
    | function y = Init_Global_State()
    | % Inizializza la struttura dello stato globale condiviso.
    | %
    | % Descrizione:
    | %   Aggrega lo stato di entrambe le schede (B1 e B2) e include flag logici
    | %   derivati necessari per l'algoritmo decisionale.
    | %
    | % Output:
    | %   - y: Struct contenente sottostrutture e flag di stato.
    | 
    |     y.stateB1 = initRecState(); % Stato della Board 1
    |     y.stateB2 = Init_State();    % Stato della Board 2
    |     
    |     % Flag logici e Enumerativi per la gestione ostacoli
    |     y.mov_obs = MOVING_OBSTACLE_TYPE.NO_OBSTACLE; 
    |     y.spc_retro = false;        % Retromarcia speciale disattivata
    |     y.limit_vel = false;        % Velocità massima
    |     y.change_vel = int8(0);     % Velocità massima
    |     y.obs_detection = true;     % Sistema anticollisione attivo
    | end
    | 
    | function y = Init_Decision()
    | % Inizializza la struttura dei comandi di attuazione.
    | %
    | % Descrizione:
    | %   Definisce i target calcolati dalla logica Stateflow da inviare agli attuatori:
    | %   riferimenti di velocità per i motori, modalità frenante, luci e stato relè e mux.
    | %
    | % Output:
    | %   - y: Struct comandi di output.
    | 
    |     % Riferimenti di velocità
    |     y.rif_FA = single(0);
    |     y.rif_FB = single(0);
    |     y.rif_BA = single(0);
    |     y.rif_BB = single(0);
    |     
    |     % Comandi freni e luci
    |     y.brk_mode = BRAKING_TYPE.NONE;
    |     y.led_A = LED_TYPE.OFF;
    |     y.led_B = LED_TYPE.OFF;
    |     y.rear_led = REAR_LED_TYPE.IDLE;
    |     y.rear_sign = REAR_SIGN_TYPE.SIGN_OFF;
    |     
    |     % Modalità operativa
    |     y.mode = ROVER_MODE.DEFAULT;
    |     y.relay = false;
    |     y.mux = false;
    | 
    | end
    |  
    | function y = Init_State_Packet()
    | % Wrapper per il pacchetto dati dello stato locale con CRC.
    | %
    | % Descrizione:
    | %   Struttura pronta per la ricezione, contenente il payload dati e 
    | %   il campo per il controllo integrità.
    | 
    |     y.state = initRecState();
    |     y.crc = uint32(0);
    | end
    | 
    | function y = Init_Global_State_Packet()
    | % Wrapper per il pacchetto dati dello stato globale con CRC.
    | %
    | % Descrizione:
    | %   Struttura pronta per la ricezione/trasmissione dello stato globale
    | %   aggregato e il relativo checksum.
    | 
    |     y.global_state = Init_Global_State();
    |     y.crc = uint32(0);
    | end
    | 
    | function y = Init_Decision_Packet()
    | % Wrapper per il pacchetto dati della decisione con CRC.
    | %
    | % Descrizione:
    | %   Struttura pronta per la ricezione/trasmissione dei comandi
    | %   di attuazione e il relativo checksum.
    | 
    |     y.decision = Init_Decision();
    |     y.crc = uint32(0);
    | end
  function Open_Session:
    | function Open_Session
    | % Imposta a livello alto (1) il segnale hardware SESSION.
    | %
    | % Descrizione:
    | %   Questa funzione marca l'inizio formale di un nuovo ciclo di supervisione.
    | %   La Board 2 (Master) alza questa linea per svegliare la Board 1 (Slave)
    | %   e indicare che sta iniziando la procedura di sincronizzazione.
    | %
    | % Dipendenze:
    | %   Richiede 'board2_functions.h' e l'implementazione C di 'IO_Set_Session'.
    | 
    |     coder.cinclude('board2_functions.h');
    |     coder.ceval('IO_Set_Session');
    | end
  function Close_Session:
    | function Close_Session
    | % Porta a livello basso (0) il segnale hardware SESSION.
    | %
    | % Descrizione:
    | %   Questa funzione sancisce la chiusura del ciclo di comunicazione corrente.
    | %   Viene chiamata dal Master in fase di inizializzazione o 
    | %   al termine della fase di Scambio Decisione (dopo aver verificato la congruenza).
    | %
    | % Dipendenze:
    | %   Richiede 'board2_functions.h' e l'implementazione C di 'reIO_Set_Session'.
    | 
    |     coder.cinclude('board2_functions.h');
    |     coder.ceval('IO_Reset_Session');
    | end
  function y = Get_Timestamp:
    | function y = Get_Timestamp
    | % Ottiene il timestamp attuale del sistema.
    | %
    | % Descrizione:
    | %   Wrapper per la funzione C 'Time_Get_Tick'. Restituisce il valore corrente
    | %   del timer di sistema. Questo valore viene salvato e utilizzato come 
    | %   punto di partenza per calcolare i timeout nelle transizioni di stato.
    | %
    | % Output:
    | %   - y: uint32 rappresentante il tempo attuale del microcontrollore (in microsecondi).
    | 
    |     coder.cinclude('board2_functions.h');
    |     y = uint32(0); % Pre-allocazione necessaria per definire il tipo uint32 per il CodeGen
    |     y = coder.ceval('Time_Get_Tick');
    | end
  function Update_Local_State:
    | function Update_Local_State
    | % Aggiorna la struttura dello stato locale con i valori correnti dei sensori.
    | %
    | % Descrizione:
    | %   Questa funzione esegue uno "snapshot" istantaneo di tutte le variabili 
    | %   di input (accelerometri, giroscopi, sonar, input utente) e le copia 
    | %   nella struttura 'state'. 
    | 
    |     coder.cinclude('board2_functions.h');
    |    
    |     % Ingresso sezione critica: Disabilita interrupt
    |     coder.ceval('OS_Enter_Critical');
    |     
    |     state.gyroYaw = gyroYaw;
    |     
    |     % --- Copia Sensori di Distanza ---
    |     state.sonar1 = sonar1;
    |     state.sonar2 = sonar2;
    |     state.sonar3 = sonar3;
    |     
    |     % --- Copia Input Utente ---
    |     state.controller_y = controller_y;
    |     state.controller_x = controller_x;
    |     state.button1 = B1;
    |     state.button2 = B2;
    |     state.button3 = B3;
    |     state.button4 = B4;
    |     state.r_stick_button = B_r_stick;
    |     state.l_stick_button = B_l_stick;
    |     state.controller_battery = controller_battery;
    | 
    |     state.controllerError = controllerError;
    |     state.gyroError = gyroError;
    |     
    |     % Uscita sezione critica: Riabilita interrupt
    |     coder.ceval('OS_Exit_Critical');
    |     
    | end
  function Wait_State:
    | function Wait_State
    | % Predispone la ricezione del pacchetto Stato Locale.
    | %
    | % Descrizione:
    | %   Configura il driver UART per ricevere i dati in arrivo e salvarli nella 
    | %   struttura 'receivedStatePacket'.
    | %
    | % Dipendenze:
    | %   Richiede 'board2_functions.h' e l'implementazione C di 'UART_Wait_State'.
    | 
    |     coder.cinclude('board2_functions.h');
    |     coder.ceval('UART_Wait_State', coder.ref(receivedStatePacket));
    | end
  function Update_Global_State:
    | function Update_Global_State
    | % Costruisce la visione globale del sistema.
    | %
    | % Descrizione:
    | %   Questa funzione aggrega le informazioni provenienti dalle due fonti 
    | %   disponibili per creare il 'Global State':
    | %   1. Dati Remoti: Estratti dal pacchetto ricevuto (receivedStatePacket).
    | %   2. Dati Locali: Presi dalla struttura 'state' appena.
    | %   3. Logica Derivata: Flag calcolati dalla logica di percezione (es. ostacoli).
    | 
    |     % Aggregazione stati hardware
    |     global_state.stateB1 = receivedStatePacket.state; % Stato ricevuto
    |     global_state.stateB2 = state;                     % Stato locale
    |     
    |     % Aggiornamento flag logici di alto livello
    |     if(moving_from_left && moving_from_right)
    |         global_state.mov_obs = MOVING_OBSTACLE_TYPE.MOVING_FROM_BOTH;
    |     elseif(moving_from_left)
    |         global_state.mov_obs = MOVING_OBSTACLE_TYPE.MOVING_FROM_LEFT;
    |     elseif(moving_from_right)
    |         global_state.mov_obs = MOVING_OBSTACLE_TYPE.MOVING_FROM_RIGHT;
    |     else
    |         global_state.mov_obs = MOVING_OBSTACLE_TYPE.NO_OBSTACLE;
    |     end
    |     global_state.spc_retro = special_retro; % Flag manovra retromarcia speciale
    |     global_state.limit_vel = limit_velocity;         % Velocità massima
    |     global_state.change_vel = change_velocity;         % Velocità massima
    |     global_state.obs_detection = obs_detection; % Stato sistema anticollisione
    |     
    | end
  function Wait_Global_State:
    | function Wait_Global_State
    | % Predispone la ricezione del pacchetto Stato Globale.
    | %
    | % Descrizione:
    | %   Configura la ricezione per il pacchetto di Global State.
    | %   I dati ricevuti verranno scritti in 'receivedGlobalStatePacket'.
    | %
    | % Dipendenze:
    | %   Richiede 'board2_functions.h' e l'implementazione C di 'UART_Wait_GlobalState'.
    | 
    |     coder.cinclude('board2_functions.h');
    |     coder.ceval('UART_Wait_GlobalState', coder.ref(receivedGlobalStatePacket));
    | end
  function Send_Local_State:
    | function Send_Local_State
    | % Avvia la trasmissione del pacchetto Stato Locale via UART.
    | %
    | % Descrizione:
    | %   Invoca la routine C che calcola il CRC, serializza la struttura 'state'
    | %   e avvia il trasferimento per l'invio.
    | %
    | % Dipendenze:
    | %   Richiede 'board2_functions.h' e l'implementazione C di 'UART_Send_Local_State'.
    | 
    |     coder.cinclude('board2_functions.h');
    |     coder.ceval('UART_Send_Local_State', coder.rref(state));
    | end
  function Wait_Decision:
    | function Wait_Decision
    | % Predispone la ricezione del pacchetto Decisione.
    | %
    | % Descrizione:
    | %   Configura la ricezione per il pacchetto contenente i comandi di attuazione.
    | %   I dati verranno salvati in 'receivedDecisionPacket'.
    | %
    | % Dipendenze:
    | %   Richiede 'board2_functions.h' e l'implementazione C di 'UART_Wait_Decision'.
    | 
    |     coder.cinclude('board2_functions.h');
    |     coder.ceval('UART_Wait_Decision', coder.ref(receivedDecisionPacket));
    | end
  function Send_Global_State:
    | function Send_Global_State
    | % Avvia la trasmissione del pacchetto Stato Globale.
    | %
    | % Descrizione:
    | %   Invia la struttura aggregata 'global_state'.
    | %
    | % Dipendenze:
    | %   Richiede 'board2_functions.h' e l'implementazione C di 'UART_Send_GlobalState'.
    | 
    |     coder.cinclude('board2_functions.h');
    |     
    |     coder.ceval('UART_Send_GlobalState', coder.rref(global_state));
    | end
  function y = Verify_State_Integrity:
    | function y = Verify_State_Integrity
    | % Verifica l'integrità del pacchetto Stato Locale ricevuto.
    | %
    | % Descrizione:
    | %   Analizza la correttezza della struttura 'receivedStatePacket'.
    | %
    | % Output:
    | %   - y: Boolean
    | %     - true: I dati sono validi.
    | %     - false: Pacchetto corrotto. 
    | %
    | % Dipendenze:
    | %   Richiede 'board2_functions.h' e l'implementazione C di 'CRC_Check_State'.
    | 
    |     coder.cinclude('board2_functions.h');
    |     y = false; % Pre-allocazione
    |     y = coder.ceval('CRC_Check_State', coder.ref(receivedStatePacket));
    | end
  function Send_Decision:
    | function Send_Decision
    | % Avvia la trasmissione del pacchetto Decisione.
    | %
    | % Descrizione:
    | %   Invia i comandi finali calcolati.
    | %
    | % Dipendenze:
    | %   Richiede 'board2_functions.h' e l'implementazione C di 'UART_Send_Decision'.
    | 
    |     coder.cinclude('board2_functions.h');
    |     
    |     coder.ceval('UART_Send_Decision', coder.rref(decision));
    | end
  function y = Verify_Global_Integrity:
    | function y = Verify_Global_Integrity
    | % Verifica l'integrità del pacchetto Stato Globale.
    | %
    | % Descrizione:
    | %   Analizza la correttezza della struttura 'receivedGlobalStatePacket'.
    | %
    | % Output:
    | %   - y: Boolean
    | %     - true: I dati sono validi.
    | %     - false: Pacchetto corrotto. 
    | %
    | % Dipendenze:
    | %   Richiede 'board2_functions.h' e l'implementazione C di 'CRC_Check_GlobalState'.
    | 
    |     coder.cinclude('board2_functions.h');
    |     y = false;
    |     y = coder.ceval('CRC_Check_GlobalState', coder.ref(receivedGlobalStatePacket));
    | end
  function Write_Output:
    | function Write_Output
    | % Scrive la decisione in output.
    | %
    | % Descrizione:
    | %   Questa funzione finalizza il ciclo di controllo trasferendo i comandi 
    | %   dalla struttura logica 'decision' alla struttura 'output'.
    | %   La variabile 'output' è l'interfaccia diretta verso i driver di basso livello
    | %   che pilotano fisicamente motori, luci e relè.
    | % Dipendenze:
    | %   Richiede 'board2_functions.h' e la gestione delle sezioni critiche.
    | 
    |     coder.cinclude('board2_functions.h');
    |     coder.ceval('OS_Enter_Critical');
    |     output = decision;
    |     coder.ceval('OS_Exit_Critical');
    |     
    | end
  function y = Verify_Decision_Integrity:
    | function y = Verify_Decision_Integrity
    | % Verifica l'integrità del pacchetto Decisione.
    | %
    | % Descrizione:
    | %   Analizza la correttezza della struttura 'receivedDecisionPacket'.
    | %
    | %
    | % Output:
    | %   - y: Boolean
    | %     - true: I dati sono validi.
    | %     - false: Pacchetto corrotto. 
    | %
    | % Dipendenze:
    | %   Richiede 'board2_functions.h' e l'implementazione C di 'CRC_Check_Decision'.
    | 
    |     coder.cinclude('board2_functions.h');
    |     y = false;
    |     y = coder.ceval('CRC_Check_Decision', coder.ref(receivedDecisionPacket));
    | end
  function y = Obs_Sonar1:
    | function y = Obs_Sonar1
    | % Verifica presenza ostacolo su Sonar 1.
    | %
    | % Descrizione:
    | %   Valuta se la lettura corrente del Sonar 1 rientra
    | %   nella finestra di distanza [MIN_DISTANCE, MAX_DISTANCE].
    | %
    | % Output:
    | %   - y: Boolean (true = ostacolo nel range valido).
    | 
    |     y = (state.sonar1 >= MIN_DISTANCE && state.sonar1 <= MAX_DISTANCE);
    |     
    | end
  function y = Obs_Sonar2:
    | function y = Obs_Sonar2
    | % Verifica presenza ostacolo su Sonar 2.
    | %
    | % Descrizione:
    | %   Valuta se la lettura corrente del Sonar 2 rientra
    | %   nella finestra di distanza [MIN_DISTANCE, MAX_DISTANCE].
    | %
    | % Output:
    | %   - y: Boolean (true = ostacolo nel range valido).    
    | 
    |     y = (state.sonar2 >= MIN_DISTANCE && state.sonar2 <= MAX_DISTANCE);
    |     
    | end
  function y = Obs_Sonar3:
    | function y = Obs_Sonar3
    | % Verifica presenza ostacolo su Sonar 3.
    | %
    | % Descrizione:
    | %   Valuta se la lettura corrente del Sonar 3 rientra
    | %   nella finestra di distanza [MIN_DISTANCE, MAX_DISTANCE].
    | %
    | % Output:
    | %   - y: Boolean (true = ostacolo nel range valido).
    | 
    |     y = (state.sonar3 >= MIN_DISTANCE && state.sonar3 <= MAX_DISTANCE);
    |     
    | end
  function y = High_Temp:
    | function y = High_Temp
    | % Predicato: Rileva condizione di Sovratemperatura.
    | %
    | % Descrizione:
    | %   Monitora la temperatura della scheda remota.
    | %   Se il valore supera la soglia di sicurezza `HIGH_TEMPERATURE`, segnala
    | %   l'anomalia.
    | %
    | % Output:
    | %   - y: Boolean (true = Temperatura eccessiva).
    | 
    |     y = receivedStatePacket.state.temperature >= HIGH_TEMPERATURE;
    |     
    | end
  function y = Low_Voltage:
    | function y = Low_Voltage
    | % Predicato: Rileva condizione di Sottotensione.
    | %
    | % Descrizione:
    | %   Controlla il livello di tensione della batteria.
    | %   Se la tensione scende sotto la soglia critica `LOW_VOLTAGE`, la funzione
    | %   restituisce true.
    | %
    | % Output:
    | %   - y: Boolean (true = Batteria scarica).
    | 
    |     y = receivedStatePacket.state.battery_voltage <= LOW_VOLTAGE;
    |     
    | end
  function y = Button1_Pressed:
    | function y = Button1_Pressed
    | % Rileva il Fronte di Salita del pulsante 1.
    | %
    | % Descrizione:
    | %   Restituisce 'true' per un singolo ciclo di esecuzione quando il pulsante
    | %   passa da rilasciato (0) a premuto (1). Ignora lo stato 'premuto fisso'.
    | %
    | % Output:
    | %   - y: Boolean (true = pulsante appena premuto).
    | 
    |     persistent prev_button1;
    |     
    |     % Inizializza la memoria al primo ciclo assoluto
    |     if isempty(prev_button1)
    |         prev_button1 = false;
    |     end
    |     
    |     % Se non siamo nel passo di esecuzione valido, esci subito.
    |     if ~STEP
    |         y = false;
    |         return;
    |     end
    |     
    |     % Leggi lo stato attuale dal bus segnali
    |     current_button1 = state.button1;
    |     
    |     % Logica Rising Edge: Attuale ALTO AND Precedente BASSO
    |     y = (current_button1 == true) && (prev_button1 == false);
    |     
    |     % Aggiorna lo stato precedente per il prossimo ciclo
    |     prev_button1 = current_button1;
    |     
    | end
  function y = Button2_Pressed:
    | function y = Button2_Pressed
    | % Rileva il Fronte di Salita del pulsante 2.
    | %
    | % Descrizione:
    | %   Restituisce 'true' per un singolo ciclo di esecuzione quando il pulsante
    | %   passa da rilasciato (0) a premuto (1). Ignora lo stato 'premuto fisso'.
    | %
    | % Output:
    | %   - y: Boolean (true = pulsante appena premuto).
    | 
    |     persistent prev_button2;
    |     
    |     % Inizializza la memoria al primo ciclo assoluto
    |     if isempty(prev_button2)
    |         prev_button2 = false;
    |     end
    |     
    |     % Se non siamo nel passo di esecuzione valido, esci subito.
    |     if ~STEP
    |         y = false;
    |         return;
    |     end
    |     
    |     % Leggi lo stato attuale dal bus segnali
    |     current_button2 = state.button2;
    |     
    |     % Logica Rising Edge: Attuale ALTO AND Precedente BASSO
    |     y = (current_button2 == true) && (prev_button2 == false);
    |     
    |     % Aggiorna lo stato precedente per il prossimo ciclo
    |     prev_button2 = current_button2;
    |     
    | end
  function y = Check_Timeout_Us(start_time, min_elapsed_time):
    | function y = Check_Timeout_Us(start_time, min_elapsed_time)
    | % Verifica se è trascorso un intervallo di tempo specifico (in microsecondi).
    | %
    | % Descrizione:
    | %   Funzione che calcola la differenza tra il tempo attuale e lo 'start_time'. 
    | %   Restituisce true solo se il delta supera 'min_elapsed_time'.
    | %   È il cuore della gestione dei timeout per l'handshake e la ricezione pacchetti.
    | %
    | % Input:
    | %   - start_time: Timestamp iniziale acquisito precedentemente con Get_Timestamp.
    | %   - min_elapsed_time: Soglia di attesa desiderata in microsecondi.
    | %
    | % Output:
    | %   - y: Boolean (true = timeout scaduto, false = tempo non ancora trascorso).
    | 
    |     coder.cinclude('board2_functions.h');
    |     y = false; % Inizializzazione tipo output (boolean)
    |     y = coder.ceval('Time_Check_Elapsed_us', start_time, min_elapsed_time);
    | end
  function y = Check_Timeout_Ms(start_time, min_elapsed_time):
    | function y = Check_Timeout_Ms(start_time, min_elapsed_time)
    | % Verifica se è trascorso un intervallo di tempo specifico (in MILLISECONDI).
    | %
    | % Descrizione:
    | %   Funzione per la gestione di timeout o ritardi nell'ordine
    | %   dei millisecondi (ms). Calcola la differenza tra il tick attuale di sistema
    | %   e lo 'start_time'. Restituisce true se il delta supera la soglia.
    | %   
    | %   A differenza di 'Check_Timeout_Us', questa variante è 
    | %   usata per logiche di decisione.
    | %
    | % Input:
    | %   - start_time: Timestamp iniziale acquisito con Get_Timestamp.
    | %   - min_elapsed_time: Durata dell'attesa desiderata in millisecondi.
    | %
    | % Output:
    | %   - y: Boolean (true = tempo scaduto, false = ancora in attesa).
    | 
    |     coder.cinclude('board2_functions.h');
    |     y = false; % Pre-allocazione del tipo boolean per il generatore di codice
    |     y = coder.ceval('Time_Check_Elapsed_ms', start_time, min_elapsed_time);
    | end
  function y = Is_STalk_High:
    | function y = Is_STalk_High
    | % Legge lo stato della linea di handshake S_TALK (Slave Talk).
    | %
    | % Descrizione:
    | %   Verifica se la Board 1 (Slave) ha alzato la sua linea di segnalazione.
    | %   Nel protocollo, un livello alto su S_TALK ha due significati principali:
    | %   1. ACK: Conferma che lo Slave ha ricevuto correttamente il pacchetto del Master.
    | %   2. READY: Indica che lo Slave è pronto a trasmettere i propri dati.
    | %
    | % Output:
    | %   - y: Boolean (true = S_TALK è alta/attiva, false = S_TALK è bassa).
    | %
    | % Dipendenze:
    | %   Chiama la funzione esterna 'IO_Read_SlaveTalk()' da 'board2_functions.h'.
    | 
    | 
    |     coder.cinclude('board2_functions.h');
    |     
    |     y = false; % Pre-allocazione per code generation
    |     y = coder.ceval('IO_Read_SlaveTalk');
    | end
  function Raise_MTalk:
    | function Raise_MTalk
    | % Imposta a livello alto (1) la linea di controllo M_TALK (Master Talk).
    | %
    | % Descrizione:
    | %   La Board 2 (Master) chiama questa funzione per asserire il controllo del bus.
    | %
    | % Dipendenze:
    | %   Richiede 'board2_functions.h' e l'implementazione C di 'IO_Set_MasterTalk'.
    | 
    |     coder.cinclude('board2_functions.h');
    |     coder.ceval('IO_Set_MasterTalk');
    | end
  function y = Is_Tx_Finished:
    | function y = Is_Tx_Finished
    | % Verifica se la trasmissione dati via UART è stata fisicamente completata.
    | %
    | % Descrizione:
    | %   Controlla se l'hardware ha finito di inviare l'ultimo bit. 
    | %
    | % Output:
    | %   - y: Boolean (true = invio completato, false = trasmissione ancora in corso).
    | 
    |     coder.cinclude('board2_functions.h');
    |     y = false; % Pre-allocazione per code generation
    |     y = coder.ceval('UART_Is_Tx_Complete');
    | end
  function y = Is_Rx_Finished:
    | function y = Is_Rx_Finished
    | % Verifica se è stato ricevuto un pacchetto dati completo via UART.
    | %
    | % Descrizione:
    | %   Funzione che interroga lo stato del driver di comunicazione.
    | %   Restituisce true quando il buffer di ricezione contiene nuovi dati pronti 
    | %   per essere letti.
    | %
    | % Output:
    | %   - y: Boolean (true = dati disponibili, false = buffer vuoto/in attesa).
    | 
    |     coder.cinclude('board2_functions.h');
    |     y = false; % Pre-allocazione per code generation
    |     y = coder.ceval('UART_Is_Rx_Complete');
    | end
  function Send_Ping:
    | function Send_Ping
    | % Invia un byte di PING via UART.
    | %
    | % Descrizione:
    | %   Spedisce un PING per testare il funzionamento della linea di UART.
    | %
    | % Dipendenze:
    | %   Richiede 'board2_functions.h' e l'implementazione C di 'UART_Send_Ping'.
    | 
    |     coder.cinclude('board2_functions.h');
    |     coder.ceval('UART_Send_Ping');
    | end
  function Wait_Ping:
    | function Wait_Ping
    | % Predispone la ricezione di un pacchetto PING.
    | %
    | % Descrizione:
    | %   Configura il driver UART per attendere il PING.
    | %   I dati ricevuti vengono salvati nella variabile 'receivedPing'.
    | %
    | % Dipendenze:
    | %   Richiede 'board2_functions.h' e l'implementazione C di 'UART_Wait_Ping'.
    | 
    |     coder.cinclude('board2_functions.h');
    |     coder.ceval('UART_Wait_Ping', coder.ref(receivedPing));
    | end
  function y = Verify_Ping:
    | function y = Verify_Ping
    | % Verifica la validità del PING ricevuto.
    | %
    | % Descrizione:
    | %   Controlla se i dati ricevuti corrispondono effettivamente la byte di
    | %   PING.
    | %
    | % Output:
    | %   - y: Boolean
    | %     - true: Ping confermato.
    | %     - false: Dati errati o rumore sulla linea.
    | %
    | % Dipendenze:
    | %   Richiede 'board2_functions.h' e l'implementazione C di 'UART_Check_Ping'.
    | 
    |     coder.cinclude('board2_functions.h');
    |     y = false;
    |     y = coder.ceval('UART_Check_Ping', receivedPing);
    | end
  function Compute_Degraded_Actions:
    | function Compute_Degraded_Actions
    | % Gestore della Logica di Controllo in Modalità Degradata.
    | %
    | % Descrizione:
    | %   Funzione esecutiva principale per la Board 2 quando opera in
    | %   isolamento.
    | %
    | % Gerarchia di Intervento (dalla più alta alla più bassa priorità):
    | %   1. CRITICITÀ ASSOLUTA: Guasto Motore o "Panic Combo".
    | %      -> Una volta attivato, richiede riavvio scheda.
    | %   2. ANTI-COLLISIONE: Arresto se ostacolo rilevato nelle vicinanze.
    | %   3. PROTEZIONE/PAUSA: Richiesta di stop controllato.
    | %   4. GUIDA MANUALE: Calcolo cinematica open-loop.
    | %
    | % Dipendenze:
    | %   Richiede 'board2_functions.h' per la gestione della sezione critica.
    | 
    |     coder.cinclude('board2_functions.h');
    |     
    |     % --- INIZIO SEZIONE CRITICA ---
    |     coder.ceval('OS_Enter_Critical');
    |     
    |     % --- VERIFICA CONDIZIONE DI BLOCCO PERMANENTE ---
    |     % Se l'utente preme la combinazione, il flag si alza e non si abbassa più.
    |     if (B1 && B2 && B3 && B4)
    |         panic_lockdown = true;
    |     end
    |     
    |     % Abilita il multiplexer
    |     output.mux = true;
    |     
    |     % Inizializzazione Default
    |     output.led_A = LED_TYPE.OFF;
    |     output.led_B = LED_TYPE.OFF;
    |     output.rear_led = REAR_LED_TYPE.IDLE;
    |     output.rear_sign = REAR_SIGN_TYPE.SIGN_OFF;
    | 
    |     % =========================================================================
    |     % LIVELLO 1: DIAGNOSTICA HARDWARE & KILL SWITCH
    |     % =========================================================================
    |     % Condizione di scatto:
    |     %   a) I driver motore segnalano un guasto interno.
    |     %   b) La variabile 'panic_lockdown' è attiva (o perché premuta ora, 
    |     %      o perché premuta in passato).
    |     if (working_status == WORKING_STATUS_TYPE.MOTOR_ERROR_WORKING) || panic_lockdown
    |         % SHUTDOWN TOTALE IMPERATIVO E PERMANENTE
    |         output.rif_FA = single(0);
    |         output.rif_FB = single(0);
    |         output.rif_BA = single(0);
    |         output.rif_BB = single(0);
    |         output.brk_mode = BRAKING_TYPE.EMERGENCY; 
    |         
    |         % Apertura del Relè di Potenza
    |         output.relay = false;
    |         
    |         % Uscita anticipata
    |         coder.ceval('OS_Exit_Critical');
    |         return; 
    |     end
    | 
    |     % =========================================================================
    |     % LIVELLO 2: SISTEMA ANTI-COLLISIONE
    |     % =========================================================================
    |     if (((sonar1 < MIN_DISTANCE) || (sonar2 < MAX_DISTANCE) || (sonar3 < MIN_DISTANCE)) ...
    |             && controller_y > CONTROLLER_ZERO)
    |         
    |         output.rif_FA = single(0);
    |         output.rif_FB = single(0);
    |         output.rif_BA = single(0);
    |         output.rif_BB = single(0);
    |         output.brk_mode = BRAKING_TYPE.EMERGENCY; 
    |         output.relay = true;
    |         
    |         coder.ceval('OS_Exit_Critical');
    |         return;
    |     end
    |     
    |     % =========================================================================
    |     % LIVELLO 3: ARRESTO DI EMERGENZA UTENTE
    |     % =========================================================================
    |     if B4        
    |         output.rif_FA = single(0);
    |         output.rif_FB = single(0);
    |         output.rif_BA = single(0);
    |         output.rif_BB = single(0);
    |         output.brk_mode = BRAKING_TYPE.EMERGENCY;
    |         output.relay = true;
    |         
    |         coder.ceval('OS_Exit_Critical');
    |         return;
    |     end
    |     
    |     % =========================================================================
    |     % LIVELLO 4: GESTIONE ENERGETICA E STOP CONTROLLATO
    |     % =========================================================================
    |     if B3 || controller_battery <= LOW_CONTROLLER_BATTERY
    |         output.rif_FA = single(0);
    |         output.rif_FB = single(0);
    |         output.rif_BA = single(0);
    |         output.rif_BB = single(0);
    |         output.brk_mode = BRAKING_TYPE.NORMAL;
    |         output.relay = true;
    |         
    |         coder.ceval('OS_Exit_Critical');
    |         return;
    |     end
    |     
    |     % =========================================================================
    |     % LIVELLO 5: OPERATIVITÀ NORMALE
    |     % =========================================================================
    |     [rif_FA, rif_FB, rif_BA, rif_BB] = Process_User_Commands_Degraded(controller_x, controller_y);
    |     
    |     output.rif_FA = rif_FA;
    |     output.rif_BA = rif_BA;
    |     output.rif_FB = rif_FB;
    |     output.rif_BB = rif_BB;
    |     
    |     output.brk_mode = BRAKING_TYPE.NONE;
    |     output.relay = true;
    |     
    |     coder.ceval('OS_Exit_Critical'); 
    |     
    | end
    | 
    | 
    | function [rif_FA, rif_FB, rif_BA, rif_BB] = Process_User_Commands_Degraded(controller_x, controller_y)
    | % Calcola i riferimenti di velocità per i 4 motori.
    | %
    | % Descrizione:
    | %   Converte gli input analogici del joystick in comandi di velocità
    | %   per i motori (RPM), applicando un algoritmo di "Arcade Drive" (miscelazione
    | %   Throttle + Steering).
    | %
    | %   Include logiche specifiche per la manovrabilità:
    | %   - Limitazione velocità massima di sicurezza (LIMITED_RPM).
    | %   - Gestione della rotazione sul posto (Pivot turn).
    | %   - Normalizzazione per mantenere il rapporto di sterzata anche a full gas.
    | %
    | % Input:
    | %   - controller_x, controller_y: Valori grezzi (0-512).
    | %
    | % Output:
    | %   - rif_FA, rif_FB, rif_BA, rif_BB: Target di velocità per i motori.
    | 
    |     % ---- 1. Configurazione Limiti ----
    |     % In modalità degradata si usa un limite conservativo
    |     MAX_SPEED = single(LIMITED_RPM);
    |     
    |     % ---- 2. Normalizzazione Input ----
    |     % Converte il range 0..512 in -1.0..+1.0 (float)
    |     diff_x = single(controller_x) - single(CENTER);
    |     diff_y = single(controller_y) - single(CENTER);
    |     
    |     steering = single(diff_x) / CENTER;  % Asse X: Sterzata (-1.0 sx, +1.0 dx)
    |     throttle = single(diff_y) / CENTER;  % Asse Y: Acceleratore (-1.0 retro, +1.0 avanti)
    | 
    |     % ---- 3. Calcolo Velocità Base ----
    |     % forward: componente lineare pura
    |     forward = throttle * MAX_SPEED;
    |     
    |     % turn: componente rotazionale pura
    |     turn = steering * MAX_SPEED;
    |     
    |     % ---- 4. Gestione Dinamica Sterzata ----
    |     if abs(throttle) < PURE_TURN_EPS
    |         % Pivot Turn: Se l'acceleratore è quasi a zero, permetti rotazione sul posto
    |         forward = single(0);
    |     else
    |         % Moving Turn: Se il rover si muove, limita la rotazione per stabilità.
    |         % La capacità di sterzare scala con la velocità lineare (TURN_RATIO).
    |         max_turn = abs(forward) * TURN_RATIO;
    |         if abs(turn) > max_turn
    |             turn = sign(turn) * max_turn;
    |         end
    |     end
    |     
    |     % ---- 5. Arcade Mixing ----
    |     % Combina movimento lineare e rotatorio per i lati sinistro e destro
    |     left  = forward + turn;
    |     right = forward - turn;
    |     
    |     % ---- 6. Normalizzazione ----
    |     % Se la somma supera il MAX_SPEED, scala entrambi i lati proporzionalmente
    |     % invece di tagliare il valore più alto. Questo preserva la curvatura
    |     % della traiettoria impostata dall'utente.
    |     maxabs = max(abs(left), abs(right));
    |     if maxabs > MAX_SPEED
    |         scale_factor = MAX_SPEED / maxabs;
    |         left  = left  * scale_factor;
    |         right = right * scale_factor;
    |     end
    |     
    |     % ---- 7. Mappatura Output ----
    |     % Assegna i valori calcolati ai 4 motori
    |     rif_FA = left;   % Front Left
    |     rif_FB = right;  % Front Right
    |     rif_BA = left;   % Back Left
    |     rif_BB = right;  % Back Right
    | end
  function Abort_Communication:
    | function Abort_Communication
    | % Sospende le operazioni di trasferimento dati UART (RX/TX).
    | %
    | % Descrizione:
    | %   Interrompe immediatamente le richieste associate alla periferica UART.
    | %
    | % Dipendenze:
    | %   Richiede 'board2_functions.h' e l'implementazione C di 'UART_DMA_Stop'.
    | 
    |     coder.cinclude('board2_functions.h');
    |     coder.ceval('UART_Stop_DMA');
    | end
  function y = Motor_Error:
    | function y = Motor_Error
    | % Verifica cumulativa di anomalie motori e input di arresto.
    | %
    | % Descrizione:
    | %   Monitora lo stato di salute dei 4 motori (Board 1) e lo stato dei 
    | %   4 pulsanti del controller (Board 2).
    | %
    | % Output:
    | %   - y: Boolean (true = Errore rilevato o Stop richiesto da pulsanti).
    | 
    |     y = (global_state.stateB1.motorError_FA || global_state.stateB1.motorError_FB || ...
    |         global_state.stateB1.motorError_BA || global_state.stateB1.motorError_BB) || ...
    |         (global_state.stateB2.button1 && global_state.stateB2.button2 && ...
    |         global_state.stateB2.button3 && global_state.stateB2.button4 || panic_lockdown);
    |     
    | end
  function y = Critical_Voltage:
    | function y = Critical_Voltage
    | % Verifica condizione di Tensione Critica.
    | %
    | % Descrizione:
    | %   Controlla se la tensione della batteria è scesa sotto la soglia di 
    | %   emergenza 'CRITICAL_VOLTAGE'.
    | %
    | % Output:
    | %   - y: Boolean (true = Tensione criticamente bassa).
    | 
    |     y = global_state.stateB1.battery_voltage <= CRITICAL_VOLTAGE;
    |     
    | end
  function y = Detect_Limit_Activation:
    | function y = Detect_Limit_Activation()
    | % Rileva l'attivazione del limitatore di velocità (Fronte di Salita).
    | %
    | % Descrizione:
    | %   Confronta lo stato corrente di 'limit_velocity' con quello memorizzato
    | %   nel ciclo precedente per identificare la transizione da FALSE a TRUE.
    | %   Utilizza una variabile 'persistent' per mantenere la memoria dello stato.
    | %   L'esecuzione è subordinata alla variabile STEP.
    | %
    | % Output:
    | %   - y: Boolean
    | %     - true:  Il segnale è appena passato da False a True (Trigger).
    | %     - false: Nessuna transizione, stato stabile o STEP non attivo.
    | 
    |     persistent prev_limit_state;
    |     
    |     % Inizializzazione della memoria al primo avvio (default false)
    |     if isempty(prev_limit_state)
    |         prev_limit_state = false;
    |     end
    |     
    |     % --- CONTROLLO EVENTO STEP ---
    |     % Se non siamo nel passo di esecuzione valido, esci subito.
    |     if ~STEP
    |         y = false;
    |         return;
    |     end
    |     
    |     % Leggi lo stato attuale dalla struttura globale
    |     current_limit_state = global_state.limit_vel;
    |     
    |     % LOGICA DI RILEVAMENTO:
    |     % Vero SE (Attuale è True) E (Precedente era False)
    |     y = current_limit_state && ~prev_limit_state;
    |     
    |     % GESTIONE MAX VELOCITY (Side Effect)
    |     if(y && (max_velocity > LIMITED_RPM))
    |         max_velocity = LIMITED_RPM;
    |     end
    |     
    |     % AGGIORNAMENTO MEMORIA:
    |     % Salva lo stato attuale per il confronto nel prossimo ciclo STEP
    |     prev_limit_state = current_limit_state;
    |     
    |     change_velocity = int8(0);
    |     
    | end
  function Increase_Max_Vel:
    | function Increase_Max_Vel
    | % Incremento controllato della soglia di velocità massima.
    | %
    | % Descrizione:
    | %   Applica un incremento a gradino (VEL_CHANGE) alla variabile 'max_vel'.
    | %   La funzione gestisce dinamicamente due tetti di saturazione diversi
    | %   in base alla modalità operativa (Normale o Limitata).
    | %   Include una protezione "Anti-Windup" per non superare mai il limite fisico
    | %   durante l'addizione.
    | %
    | % Output:
    | %   - max_vel: Aggiornato e saturato al limite attivo (MAX_RPM o LIMITED_RPM).
    | 
    |     % ---- 1. Selezione del limite attivo ----
    |     if global_state.limit_vel
    |         current_limit = LIMITED_RPM;
    |     else
    |         current_limit = MAX_RPM;
    |     end
    |     % ---- 2. Applicazione Incremento e Saturazione ----
    |     % Calcola il potenziale nuovo valore
    |     next_vel = max_velocity + VEL_CHANGE;
    |     % Assegna il minimo tra il valore calcolato e il limite.
    |     if next_vel > current_limit
    |         max_velocity = current_limit;
    |     else
    |         max_velocity = next_vel;
    |     end
    | 
    |     change_velocity = int8(0);
    |     
    | end
  function Decrease_Max_Vel:
    | function Decrease_Max_Vel
    | % Decremento controllato della soglia di velocità massima.
    | %
    | % Descrizione:
    | %   Applica un decremento a gradino (VEL_CHANGE) alla variabile 'max_vel'.
    | %   Include una protezione di "Saturazione Inferiore" per garantire che
    | %   il valore non scenda mai sotto il limite fisico (MIN_RPM).
    | %
    | % Output:
    | %   - max_vel: Aggiornato e saturato a MIN_RPM se necessario.
    | 
    |     % ---- 1. Calcolo del potenziale nuovo valore ----
    |     next_vel = max_velocity - VEL_CHANGE;
    |     
    |     % ---- 2. Controllo Limiti e Saturazione ----
    |     % Se il nuovo valore calcolato è inferiore al minimo consentito,
    |     % forziamo la variabile al minimo (MIN_RPM).
    |     
    |     if next_vel < MIN_RPM
    |         max_velocity = MIN_RPM;
    |     else
    |         max_velocity = next_vel;
    |     end
    | 
    |     change_velocity = int8(0);
    |     
    | end
  function Stop_Motors:
    | function Stop_Motors
    | % Imposta i riferimenti di velocità a ZERO per tutti i motori.
    | %
    | % Descrizione:
    | %   Azzera i comandi di velocità per i quattro motori (Front/Back, Lato A/B).
    | 
    |     decision.rif_FA = single(0);
    |     decision.rif_FB = single(0);
    |     decision.rif_BA = single(0);
    |     decision.rif_BB = single(0);
    | 
    | end
  function Process_Evasive_Commands(turn_right, opn_loop):
    | function Process_Evasive_Commands(turn_right, opn_loop)
    | % Implementa l'algoritmo di guida per evitamento ostacoli in movimento.
    | %
    | % Descrizione:
    | %   Calcola i riferimenti di velocità per le ruote combinando l'input
    | %   di avanzamento (Controller Y) con una sterzata evasiva forzata.
    | %
    | % Input:
    | %   - turn_right: (Boolean/Flag)
    | %       true  -> Impone sterzata a DESTRA (Steering +1)
    | %       false -> Impone sterzata a SINISTRA (Steering -1)
    | 
    | 
    |     % ---- Parametri ----
    |     if(opn_loop)
    |         MAX_SPEED = single(LIMITED_RPM);
    |     else
    |         MAX_SPEED = single(max_velocity);
    |     end
    | 
    |     % ---- Input Controller (Y) ----
    |     % Calcola la richiesta di avanzamento basandosi sullo stick analogico
    |     diff_y   = single(global_state.stateB2.controller_y) - single(CENTER);
    |     throttle = diff_y / single(CENTER);    % Range normalizzato: [-1 .. +1]
    | 
    |     % ---- Direzione evasiva ----
    |     % La direzione di sterzata è determinata dall'argomento in ingresso.
    |     if turn_right
    |         steering_dir = single(+1); % Rotazione oraria (Destra)
    |     else
    |         steering_dir = single(-1); % Rotazione antioraria (Sinistra)
    |     end
    |     
    |     % ---- Velocità base ----
    |     forward = throttle * MAX_SPEED;
    | 
    |     % ---- Steering dinamico ----
    |     % Aumenta l'aggressività della sterzata se il rover si muove più velocemente
    |     turn_scale = MIN_TURN_SCALE_EVASIVE + ...
    |                  (MAX_TURN_SCALE_EVASIVE - MIN_TURN_SCALE_EVASIVE) * abs(throttle);
    |     
    |     % Calcolo componente di rotazione grezza
    |     turn = steering_dir * MAX_SPEED * turn_scale;
    | 
    |     % ---- Limitazione dinamica della sterzata ----
    |     % Se il rover è in movimento (throttle > soglia), limita la rotazione
    |     % per evitare testacoda o instabilità (mantieni rapporto con forward).
    |     if abs(throttle) >= PURE_TURN_EPS
    |         max_turn = abs(forward) * TURN_RATIO;
    |         if abs(turn) > max_turn
    |             turn = sign(turn) * max_turn;
    |         end
    |     end
    | 
    |     % ---- Mixing differenziale ----
    |     % Calcola velocità sinistra/destra
    |     left  = forward + turn;
    |     right = forward - turn;
    | 
    |     % ---- Normalizzazione ----
    |     % Se i valori superano la velocità massima fisica, scala entrambi
    |     % proporzionalmente per mantenere la traiettoria (curvatura) corretta.
    |     maxabs = max(abs(left), abs(right));
    |     if maxabs > MAX_SPEED
    |         scale_factor = MAX_SPEED / maxabs;
    |         left  = left  * scale_factor;
    |         right = right * scale_factor;
    |     end
    | 
    |     % ---- Output ----
    |     decision.rif_FA = left;
    |     decision.rif_BA = left;
    |     decision.rif_FB = right;
    |     decision.rif_BB = right;
    | end
  function Process_User_Commands(opn_loop):
    | function Process_User_Commands(opn_loop)
    | % Implementa l'algoritmo di guida (Miscelazione Throttle + Steering).
    | %
    | % Descrizione:
    | %   Trasforma gli input grezzi del joystick in riferimenti 
    | %   di velocità per i 4 motori (RPM).
    | 
    |     % ---- 1. Selezione profilo di velocità ----
    |     if(opn_loop)
    |         MAX_SPEED = single(LIMITED_RPM);
    |     else
    |         MAX_SPEED = single(max_velocity);
    |     end
    |     
    |     % ---- 2. Conversione e Normalizzazione Input ----
    |     % Converte il range del controller [0..512] in un range normalizzato [-1.0..+1.0].
    |     diff_x = single(global_state.stateB2.controller_x) - single(CENTER);
    |     diff_y = single(global_state.stateB2.controller_y) - single(CENTER);
    |     
    |     steering = single(diff_x) / CENTER;  % Asse X: -1.0 (Sinistra) .. +1.0 (Destra)
    |     throttle = single(diff_y) / CENTER;  % Asse Y: -1.0 (Indietro) .. +1.0 (Avanti)
    | 
    |     % ---- 3. Calcolo velocità base ----
    |     % Mappa gli input normalizzati sul range di RPM fisico.
    |     
    |     % Componente Lineare (Forward): Dipende esclusivamente dalla levetta Y.
    |     forward = throttle * MAX_SPEED;
    |     
    |     % Componente Angolare (Turn): Potenziale di rotazione basato sulla levetta X.
    |     turn = steering * MAX_SPEED;
    |     
    |     % ---- 4. Gestione dinamica della sterzata ----
    |     if abs(throttle) < PURE_TURN_EPS
    |         % CASO A: Rotazione sul posto.
    |         forward = single(0); % Forza velocità lineare a zero per evitare drift
    |     else
    |         % CASO B: Curva in movimento.
    |         % Limita l'autorità di sterzata in funzione della velocità di avanzamento.
    |         max_turn = abs(forward) * TURN_RATIO;
    |         if abs(turn) > max_turn
    |             turn = sign(turn) * max_turn;
    |         end
    |     end
    |     
    |     % ---- 5. Mixing Differenziale ----
    |     left  = forward + turn;
    |     right = forward - turn;
    |     
    |     % ---- 6. Normalizzazione Proporzionale ----
    |     % CRITICO: Se la somma (Forward + Turn) supera il MAX_SPEED fisico,
    |     % non possiamo semplicemente tagliare (clamping) il valore eccedente,
    |     % altrimenti il robot cambierebbe raggio di curvatura.
    |     %
    |     % Soluzione: Scaliamo ENTRAMBI i lati dello stesso fattore per mantenere
    |     % il rapporto L/R costante (e quindi la traiettoria curva corretta),
    |     % riducendo la velocità complessiva.
    |     maxabs = max(abs(left), abs(right));
    |     if maxabs > MAX_SPEED
    |         scale_factor = MAX_SPEED / maxabs;
    |         left  = left  * scale_factor;
    |         right = right * scale_factor;
    |     end
    |     
    |     % ---- 7. Assegnazione Output ai 4 Motori ----
    |     decision.rif_FA = left;
    |     decision.rif_BA = left;
    |     decision.rif_FB = right;
    |     decision.rif_BB = right;
    |     
    | end
  function Turn_Right:
    | function Turn_Right
    | % Esegue una rotazione sul posto verso DESTRA.
    | %
    | % Descrizione:
    | %   Configura i motori in modalità contro-rotante per girare in senso orario.
    | %   - Lato Sinistro (A): Spinge in Avanti (+).
    | %   - Lato Destro (B): Tira Indietro (-).
    | 
    |     decision.rif_FA = TURN_RPM;
    |     decision.rif_FB = -TURN_RPM;
    |     decision.rif_BA = TURN_RPM;
    |     decision.rif_BB = -TURN_RPM;
    | 
    | end
  function Turn_Left:
    | function Turn_Left
    | % Esegue una rotazione sul posto verso SINISTRA.
    | %
    | % Descrizione:
    | %   Configura i motori in modalità contro-rotante per girare in senso antiorario.
    | %   - Lato Sinistro (A): Tira Indietro (-).
    | %   - Lato Destro (B): Spinge in Avanti (+).
    | 
    |     decision.rif_FA = -TURN_RPM;
    |     decision.rif_FB = TURN_RPM;
    |     decision.rif_BA = -TURN_RPM;
    |     decision.rif_BB = TURN_RPM;
    | 
    | end
  function Turn_Back:
    | function Turn_Back
    | % Esegue una manovra di Inversione rapida.
    | %
    | % Descrizione:
    | %   Configura i motori per effettuare una retromarcia normale.
    | 
    |     decision.rif_FA = TURN_BACK_RPM;
    |     decision.rif_FB = -TURN_BACK_RPM;
    |     decision.rif_BA = TURN_BACK_RPM;
    |     decision.rif_BB = -TURN_BACK_RPM;
    |     
    | end
  function Update_Angle(yaw):
    | function Update_Angle(yaw)
    | % Aggiorna la stima dell'angolo tramite Integrazione.
    | %
    | % Descrizione:
    | %   Implementa l'Integrazione Numerica col "Metodo dei Trapezi".
    | %   Converte la velocità angolare (giroscopio) n un angolo assoluto 
    | %   accumulato nel tempo.
    | %
    | %   Formula:
    | %   Angle(t) = Angle(t-1) + 0.5 * (Rate(t) + Rate(t-1)) * dT
    | %
    | % Input:
    | %   - yaw: Velocità angolare corrente [deg/s].
    | 
    |     angle = angle + 0.5 * (yaw + prevYaw) * PERIOD;
    |     prevYaw = yaw;
    | 
    | end
  function y = Is_Rover_Moving_Forward:
    | function y = Is_Rover_Moving_Forward
    | % Verifica cinematica: Il Rover sta avanzando?
    | %
    | % Descrizione:
    | %   Analizza il feedback di velocità reale dai motori.
    | %   Serve per confermare che il rover stia eseguendo un movimento in
    | %   avanti.
    | %
    | % Output:
    | %   - y: Boolean
    | %     - true: Tutte e 4 le ruote hanno velocità positiva (> 0).
    | %     - false: Altrimenti.
    | 
    |     velocities = [
    |         global_state.stateB1.velocity_FA
    |         global_state.stateB1.velocity_FB
    |         global_state.stateB1.velocity_BA
    |         global_state.stateB1.velocity_BB
    |     ];
    |     
    |     y = all(velocities > STOP_THRESHOLD);
    | 
    | end
  function y = Emergency_B_Routine:
    | function y = Emergency_B_Routine
    | % Routine di Frenata di Emergenza (Button 4).
    | %
    | % Descrizione:
    | %   Attiva la procedura di emergenza su richiesta dell'operatore.
    | %
    | % Output:
    | %   - y: Boolean (true = Avviare routine emergenza manuale).
    | 
    |     y = STEP && (global_state.stateB2.button4 && ...
    |         global_state.stateB2.controller_battery > LOW_CONTROLLER_BATTERY);
    | 
    | end
  function y = Emergency_S_Routine:
    | function y = Emergency_S_Routine
    | % Routine di Emergenza Sonar.
    | %
    | % Descrizione:
    | %   Monitora i sensori ultrasonici per rilevare ostacoli a distanza critica
    | %   che richiedono un arresto istantaneo per evitare l'impatto.
    | %
    | % Output:
    | %   - y: Boolean (true = Pericolo immediato).
    | 
    |     % Selezione soglia in base allo stato dell'obstacle detection
    |     if global_state.obs_detection
    |         distance_threshold = IMM_DISTANCE;   % cm
    |     else
    |         distance_threshold = PROTECTION_DISTANCE;   % cm
    |     end
    | 
    |     y = STEP && ...
    |         (global_state.stateB2.sonar1 <= distance_threshold || ...
    |          global_state.stateB2.sonar2 <= distance_threshold || ...
    |          global_state.stateB2.sonar3 <= distance_threshold) && ...
    |         Is_Rover_Moving_Forward();
    | 
    | end
  function y = Mov_Obs_R_Routine:
    | function y = Mov_Obs_R_Routine
    | % Gestione Ostacolo Mobile da DESTRA.
    | %
    | % Descrizione:
    | %   Rileva la presenza di un oggetto dinamico che sta attraversando 
    | %   la traiettoria provenendo da destra.
    | %
    | % Output:
    | %   - y: Boolean (true = Avviare manovra di evitamento per ostacolo da Dx).
    | 
    |     y = STEP && (global_state.mov_obs == MOVING_OBSTACLE_TYPE.MOVING_FROM_RIGHT && ...
    |         Is_Rover_Moving_Forward() && global_state.obs_detection);
    | end
  function y = Mov_Obs_L_Routine:
    | function y = Mov_Obs_L_Routine
    | % Gestione Ostacolo Mobile da SINISTRA.
    | %
    | % Descrizione:
    | %   Analogo a 'Mov_Obs_R_Routine', ma gestisce gli oggetti che tagliano la strada
    | %   provenendo da sinistra.
    | %   
    | % Output:
    | %   - y: Boolean (true = Avviare manovra per ostacolo da Sx).
    | 
    |     y = STEP && (global_state.mov_obs == MOVING_OBSTACLE_TYPE.MOVING_FROM_LEFT && ...
    |         Is_Rover_Moving_Forward() && global_state.obs_detection);
    | end
  function y = Stop_Slow_Routine:
    | function y = Stop_Slow_Routine
    | % Routine di Stop Controllato.
    | %
    | % Descrizione:
    | %   Attiva una modalità di arresto cauto.
    | %
    | % Output:
    | %   - y: Boolean (true = Attiva stop dolce).
    | 
    |     y = STEP && (((global_state.stateB2.sonar2 <= MAX_DISTANCE || ...
    |         global_state.mov_obs == MOVING_OBSTACLE_TYPE.MOVING_FROM_BOTH) && ...
    |         Is_Rover_Moving_Forward() && global_state.obs_detection)  || ...
    |         (global_state.stateB2.button3 && global_state.stateB2.controller_battery > LOW_CONTROLLER_BATTERY) || ...
    |         (global_state.stateB2.controllerError));
    | end
  function y = Low_Controller_Battery_Routine:
    | function y = Low_Controller_Battery_Routine
    | % Fail-Safe Batteria Radiocomando.
    | %
    | % Descrizione:
    | %   Monitora lo stato di carica del controller remoto (Joystick).
    | %
    | % Output:
    | %   - y: Boolean (true = Batteria telecomando critica).
    | 
    |     y = STEP && (global_state.stateB2.controller_battery <= LOW_CONTROLLER_BATTERY);
    | 
    | end
  function y = Spec_Retro_Routine:
    | function y = Spec_Retro_Routine
    | % Routine Retromarcia Speciale.
    | %
    | % Descrizione:
    | %   Rileva l'intenzione dell'utente di entrare in una modalità di retromarcia
    | %   speciale.
    | %
    | % Output:
    | %   - y: Boolean (true = Avvia manovra speciale indietro).
    | 
    |     y = STEP && (global_state.stateB2.controller_y < CONTROLLER_ZERO) && ...
    |         global_state.spc_retro && ~open_loop;
    | 
    | end
  function y = Stationary_Obs_Routine:
    | function y = Stationary_Obs_Routine
    | % Inibizione alla Partenza.
    | %
    | % Descrizione:
    | %   Impedisce al rover di muoversi da fermo se c'è un ostacolo direttamente davanti.
    | %
    | % Output:
    | %   - y: Boolean (true = Rifiuta comando di avanzamento).
    | 
    |     y = STEP && Is_Rover_Stationary() && global_state.stateB2.sonar2 <= MAX_DISTANCE && ...
    |         global_state.stateB2.controller_y > CONTROLLER_ZERO && global_state.obs_detection;
    | 
    | end
  function y = Emergency_B_Pressed:
    | function y = Emergency_B_Pressed
    | % Rileva la pressione del Pulsante di Emergenza.
    | %
    | % Descrizione:
    | %   Monitora il Button 4. Include un controllo di integrità sul segnale (Battery Check).
    | %
    | % Output:
    | %   - y: Boolean (true = E-Stop richiesto manualmente).
    | 
    |     y = STEP && (global_state.stateB2.button4 && ...
    |         global_state.stateB2.controller_battery > LOW_CONTROLLER_BATTERY);
    | 
    | end
  function y = Stop_B_Pressed:
    | function y = Stop_B_Pressed
    | % Rileva la richiesta di Stop Operativo (Button 3).
    | %
    | % Descrizione:
    | %   Monitora il Button 3. Viene applicato il controllo sulla validità della batteria
    | %   del trasmettitore.
    | %
    | % Output:
    | %   - y: Boolean (true = Stop operativo richiesto).
    | 
    |     y = STEP && (global_state.stateB2.button3 && ...
    |         global_state.stateB2.controller_battery > LOW_CONTROLLER_BATTERY);
    | end
  function y = Near_Obstacle:
    | function y = Near_Obstacle
    | % Rileva Ostacolo nelle vicinanze.
    | %
    | % Descrizione:
    | %   Verifica se un qualsiasi oggetto si trova entro la distanza critica 
    | %   su uno dei tre fronti (Sx, Centro, Dx).
    | %
    | % Output:
    | %   - y: Boolean (true = Oggetto troppo vicino).
    | 
    |     % Selezione soglia in base allo stato dell'obstacle detection
    |     if global_state.obs_detection
    |         distance_threshold = IMM_DISTANCE;   % cm
    |     else
    |         distance_threshold = PROTECTION_DISTANCE;   % cm
    |     end
    | 
    |     y = STEP && ...
    |         (global_state.stateB2.sonar1 <= distance_threshold || ...
    |          global_state.stateB2.sonar2 <= distance_threshold || ...
    |          global_state.stateB2.sonar3 <= distance_threshold);
    | end
  function y = Mov_Obs_Right:
    | function y = Mov_Obs_Right
    | % Classificazione Ostacolo Mobile da DESTRA.
    | %
    | % Descrizione:
    | %   Verifica se il sistema di percezione ha classificato l'oggetto attualmente 
    | %   tracciato come "in arrivo da Destra".
    | %
    | % Output:
    | %   - y: Boolean (true = Rilevato ostacolo dinamico proveniente da Dx).
    | 
    |     y = STEP && (global_state.mov_obs == MOVING_OBSTACLE_TYPE.MOVING_FROM_RIGHT ...
    |         && global_state.obs_detection);
    | 
    | end
  function y = Mov_Obs_Left:
    | function y = Mov_Obs_Left
    | % Classificazione Ostacolo Mobile da SINISTRA.
    | %
    | % Descrizione:
    | %   Verifica se il sistema di percezione ha classificato l'oggetto attualmente 
    | %   tracciato come "in arrivo da Sinistra".
    | %
    | % Output:
    | %   - y: Boolean (true = Rilevato ostacolo dinamico proveniente da Sx).
    | 
    |     y = STEP && (global_state.mov_obs == MOVING_OBSTACLE_TYPE.MOVING_FROM_LEFT ...
    |         && global_state.obs_detection);
    | 
    | end
  function y = Mode_B_Pressed:
    | function y = Mode_B_Pressed
    | % Rileva il Fronte di Salita del pulsante di Cambio Modalità.
    | %
    | % Descrizione:
    | %   Monitora il pulsante integrato nello stick analogico sinistro del
    | %   controller.
    | %
    | % Output:
    | %   - y: Boolean (true = Click stick sinistro appena rilevato).
    | 
    |     persistent prev_l_stick_button;
    |     
    |     % Inizializza al primo ciclo
    |     if isempty(prev_l_stick_button)
    |         prev_l_stick_button = false;
    |     end
    |     
    |     % Esegui solo se il passo di calcolo è attivo
    |     if ~STEP
    |         y = false;
    |         return;
    |     end
    |     
    |     % Leggi lo stato attuale dalla struttura globale consolidata
    |     current_l_stick_button = global_state.stateB2.l_stick_button;
    |     
    |     % Rileva fronte di salita (Rising Edge)
    |     y = (current_l_stick_button == true) && (prev_l_stick_button == false);
    |     
    |     % Aggiorna memoria per il ciclo successivo
    |     prev_l_stick_button = current_l_stick_button;
    |     
    | end
  function y = Is_Rover_Stationary:
    | function y = Is_Rover_Stationary
    | % Verifica cinematica: Il Rover è fisicamente fermo?
    | %
    | % Descrizione:
    | %   Questa funzione conferma se le ruote sono effettivamente ferme.
    | %
    | % Output:
    | %   - y: Boolean
    | %     - true: Tutte e 4 le ruote hanno velocità rilevata pari a 0.
    | %     - false: Almeno una ruota si sta muovendo.
    | 
    |     velocities = [
    |         global_state.stateB1.velocity_FA
    |         global_state.stateB1.velocity_FB
    |         global_state.stateB1.velocity_BA
    |         global_state.stateB1.velocity_BB
    |     ];
    |     
    |     y = all(abs(velocities) <= STOP_THRESHOLD);
    | 
    | end
  function y = Motor_Error_Occured:
    | function y = Motor_Error_Occured
    | % Verifica cumulativa degli errori motore.
    | %
    | % Descrizione:
    | %   Controlla i flag di errore individuali per tutti e quattro i motori
    | %   (Anteriore/Posteriore, Lato A/B). La funzione agisce come un "OR" logico:
    | %   basta che un solo motore sia in errore per attivare l'allarme.
    | %
    | % Output:
    | %   - y: Boolean (true = Almeno un motore ha segnalato un errore).
    | 
    |     y = working_status == WORKING_STATUS_TYPE.MOTOR_ERROR_WORKING;
    |     
    | end
  function y = Critical_Voltage_Occured:
    | function y = Critical_Voltage_Occured
    | % Verifica condizione di Tensione Critica.
    | %
    | % Descrizione:
    | %   Controlla se la tensione della batteria è scesa sotto la soglia di 
    | %   emergenza 'CRITICAL_VOLTAGE'.
    | %
    | % Output:
    | %   - y: Boolean (true = Tensione criticamente bassa).
    | 
    |     y = working_status == WORKING_STATUS_TYPE.CRITICAL_VOLTAGE_WORKING;
    |     
    | end
  function Rover_Lights_OFF:
    | function Rover_Lights_OFF
    | % Spegne tutte le luci del Rover (Stato Idle).
    | %
    | % Descrizione:
    | %   Porta tutti gli indicatori luminosi (LED anteriori, posteriori e strip)
    | %   nello stato di spegnimento.
    | 
    |     decision.led_A = LED_TYPE.OFF;
    |     decision.led_B = LED_TYPE.OFF;
    |     decision.rear_led = REAR_LED_TYPE.IDLE;
    |     decision.rear_sign = REAR_SIGN_TYPE.SIGN_OFF;
    | 
    | end
  function Rover_Lights_Motor_Error:
    | function Rover_Lights_Motor_Error
    | % Imposta la segnalazione luminosa per un errore dei motori.
    | %
    | % Descrizione:
    | %   Configura gli indicatori visivi del rover per segnalare uno stato di
    | %   guasto ai motori.
    | %   - LED Anteriori (A/B): Rosso lampeggiante per massima allerta.
    | %   - Luci Posteriori: Luce di stop e segnale rosso per indicare il fermo macchina.
    | 
    |     decision.led_A = LED_TYPE.BLINKING_RED_SLOW;
    |     decision.led_B = LED_TYPE.BLINKING_RED_SLOW;
    |     decision.rear_led = REAR_LED_TYPE.EMERGENCY_LIGHTS;
    |     decision.rear_sign = REAR_SIGN_TYPE.SIGN_RED;
    | 
    | end
  function Update_Rover_Lights(white_led_when_stopped):
    | function Update_Rover_Lights(white_led_when_stopped)
    | % Gestore centrale della logica di illuminazione.
    | %
    | % Descrizione:
    | %   Determina lo stato dei LED (Frontali, Posteriori e Cartello) basandosi 
    | %   sulla cinematica corrente e sulla modalità operativa del veicolo.
    | %   Implementa una macchina a stati a priorità decrescente per le luci di segnalazione.
    | %
    | % Logica di Priorità (dalla più alta alla più bassa):
    | %   1. ROTAZIONE SPECIALE: Segnala manovra speciale.
    | %   2. FRENATA: Segnala arresto.
    | %   3. ROTAZIONE (Pivot): Segnala manovra sul posto.
    | %   4. STERZATA (Curve): Segnala svolta in avanzamento.
    | %   5. RETROMARCIA: Luci bianche posteriori.
    | %   6. MARCIA AVANTI / STOP: Luci di posizione standard.
    | %
    | % Argomenti:
    | %   - white_led_when_stopped: Configurazione utente.
    | %     - true: Luci di posizione anteriori accese anche da fermo.
    | %     - false: Luci anteriori spente a motore fermo.
    |     
    |     if Is_Rover_In_Special_Rotation()
    |         % PRIORITY 1: Rotazione Speciale
    |         decision.led_A = LED_TYPE.BLINKING_WHITE;
    |         decision.led_B = LED_TYPE.BLINKING_WHITE;
    |         decision.rear_led = REAR_LED_TYPE.SPECIAL_LIGHTS;
    |         
    |     elseif Is_Rover_Braking()
    |         % PRIORITY 2: Frenata
    |         decision.led_A = LED_TYPE.WHITE;
    |         decision.led_B = LED_TYPE.WHITE;
    |         decision.rear_led = REAR_LED_TYPE.BRAKING_LIGHTS;
    |         
    |     elseif Is_Rover_Rotating_Left()
    |         % PRIORITY 3: Rotazione sul posto Sinistra
    |         decision.led_A = LED_TYPE.BLINKING_RED;
    |         decision.led_B = LED_TYPE.WHITE;
    |         decision.rear_led = REAR_LED_TYPE.ARROW_LEFT;
    |         
    |     elseif Is_Rover_Rotating_Right()
    |         % PRIORITY 3: Rotazione sul posto Destra
    |         decision.led_A = LED_TYPE.WHITE;
    |         decision.led_B = LED_TYPE.BLINKING_RED; 
    |         decision.rear_led = REAR_LED_TYPE.ARROW_RIGHT;
    |         
    |     elseif Is_Rover_Moving_Forward_Left()
    |         % PRIORITY 4: Curva in avanzamento Sinistra
    |         decision.led_A = LED_TYPE.BLINKING_RED;
    |         decision.led_B = LED_TYPE.WHITE;
    |         decision.rear_led = REAR_LED_TYPE.ARROW_LEFT;
    |         
    |     elseif Is_Rover_Moving_Forward_Right()
    |         % PRIORITY 4: Curva in avanzamento Destra
    |         decision.led_A = LED_TYPE.WHITE;
    |         decision.led_B = LED_TYPE.BLINKING_RED;
    |         decision.rear_led = REAR_LED_TYPE.ARROW_RIGHT;
    |         
    |     elseif Is_Rover_Moving_Backward()
    |         % PRIORITY 5: Retromarcia
    |         decision.led_A = LED_TYPE.WHITE;
    |         decision.led_B = LED_TYPE.WHITE;
    |         decision.rear_led = REAR_LED_TYPE.BACKWARD_LIGHTS;
    |        
    |     elseif Is_Rover_Moving_Forward()
    |         % PRIORITY 6: Marcia Avanti
    |         decision.led_A = LED_TYPE.WHITE;
    |         decision.led_B = LED_TYPE.WHITE;
    |         decision.rear_led = REAR_LED_TYPE.BACKLIGHTS;
    |     else
    |         % PRIORITY 7: Veicolo Fermo
    |         if white_led_when_stopped
    |             decision.led_A = LED_TYPE.WHITE;
    |             decision.led_B = LED_TYPE.WHITE;
    |         else
    |             decision.led_A = LED_TYPE.OFF;
    |             decision.led_B = LED_TYPE.OFF;
    |         end
    |         decision.rear_led = REAR_LED_TYPE.BACKLIGHTS;
    |     end
    |     
    |     % ---- 2. Aggiornamento Cartello Posteriore ----
    |     decision.rear_sign = Get_Rear_Sign_Color();
    | 
    | end
    | 
    | function y = Is_Rover_In_Special_Rotation()
    | % Rileva se è attiva la modalità di rotazione speciale.
    | %
    | % Output:
    | %   - y: Boolean 
    | %     - true: Manovra speciale attiva.
    | %     - false: Nessuna manovra speciale in corso.
    | 
    |     y = special_retro_rotating;
    | end
    | 
    | 
    | function y = Is_Rover_Braking()
    | % Rileva se il sistema frenante è attivo.
    | %
    | % Output:
    | %   - y: Boolean 
    | %     - true: È richiesto un freno. Le luci stop devono accendersi.
    | %     - false: Nessuna frenata attiva.
    | 
    |     y = decision.brk_mode ~= BRAKING_TYPE.NONE;
    | end
    |             
    | function y = Is_Rover_Rotating_Left()
    | % Rileva rotazione antioraria sul posto.
    | %
    | % Output:
    | %   - y: Boolean 
    | %     - true: Rotazione SX. Il rover gira su se stesso (SX indietro, DX avanti).
    | %     - false: Altro tipo di movimento.
    | 
    |     left_ref = (decision.rif_FA + decision.rif_BA) / 2;
    |     right_ref = (decision.rif_FB + decision.rif_BB) / 2;
    |     
    |     y = (left_ref < -STOP_THRESHOLD) && (right_ref > STOP_THRESHOLD);
    | end
    | 
    | function y = Is_Rover_Rotating_Right()
    | % Rileva rotazione oraria sul posto (Tank Turn).
    | %
    | % Output:
    | %   - y: Boolean
    | %     - true: Rotazione DX. Il rover gira su se stesso (SX avanti, DX indietro).
    | %     - false: Altro tipo di movimento.
    | 
    |     left_ref = (decision.rif_FA + decision.rif_BA) / 2;
    |     right_ref = (decision.rif_FB + decision.rif_BB) / 2;
    |     
    |     y = (left_ref > STOP_THRESHOLD) && (right_ref < -STOP_THRESHOLD);
    | end
    | 
    | function y = Is_Rover_Moving_Forward()
    | % Rileva avanzamento rettilineo puro.
    | %
    | % Output:
    | %   - y: Boolean
    | %     - true: Marcia avanti dritta. Tutti i motori hanno velocità positiva e identica.
    | %     - false: Altro tipo di movimento.
    | 
    |     fa = decision.rif_FA;
    |     fb = decision.rif_FB;
    |     ba = decision.rif_BA;
    |     bb = decision.rif_BB;
    |     
    |     references = [fa fb ba bb];
    |     
    |     y = all(references > STOP_THRESHOLD) && ...
    |         (fa == fb) && (fa == ba) && (fa == bb);
    | end
    | 
    | function y = Is_Rover_Moving_Forward_Left()
    | % Rileva sterzata differenziale a sinistra in avanzamento.
    | %
    | % Output:
    | %   - y: Boolean
    | %     - true: Curva a SX. Il rover avanza, ma il lato destro è significativamente più veloce 
    | %             del sinistro (oltre la soglia TURN_THRESHOLD).
    | %     - false: Rettilineo o curva non significativa.
    | 
    |     left_ref = (decision.rif_FA + decision.rif_BA) / 2;
    |     right_ref = (decision.rif_FB + decision.rif_BB) / 2;
    |     
    |     y = (left_ref > STOP_THRESHOLD) && ...
    |         (right_ref > STOP_THRESHOLD) && ...
    |         ((right_ref - left_ref) > TURN_THRESHOLD);
    | end
    | 
    | function y = Is_Rover_Moving_Forward_Right()
    | % Rileva sterzata differenziale a destra in avanzamento.
    | %
    | % Output:
    | %   - y: Boolean
    | %     - true: Curva a DX. Il rover avanza, ma il lato sinistro è significativamente più veloce
    | %             del destro (oltre la soglia TURN_THRESHOLD).
    | %     - false: Rettilineo o curva non significativa.
    | 
    |     left_ref = (decision.rif_FA + decision.rif_BA) / 2;
    |     right_ref = (decision.rif_FB + decision.rif_BB) / 2;
    |     
    |     y = (left_ref > STOP_THRESHOLD) && ...
    |         (right_ref > STOP_THRESHOLD) && ...
    |         ((left_ref - right_ref) > TURN_THRESHOLD);
    | end
    | 
    | function y = Is_Rover_Moving_Backward()
    | % Rileva marcia indietro (Retromarcia).
    | %
    | % Output:
    | %   - y: Boolean
    | %     - true: Retromarcia attiva. Tutti i riferimenti ai motori sono negativi.
    | %     - false: Il rover è fermo o avanza.
    | 
    |     references = [
    |         decision.rif_FA
    |         decision.rif_FB
    |         decision.rif_BA
    |         decision.rif_BB
    |     ];
    |     
    |     y = all(references < -STOP_THRESHOLD);
    |     
    | end
    | 
    | 
    | function color = Get_Rear_Sign_Color()
    | % Determina la configurazione cromatica del pannello posteriore.
    | %
    | % Descrizione:
    | %   Effettua il mapping tra la modalità operativa corrente del rover
    | %   e il codice colore da visualizzare sul display LED posteriore. 
    | %   Serve a comunicare visivamente lo stato del sistema agli operatori esterni.
    | %
    | % Output:
    | %   - color: Enum (REAR_SIGN_TYPE)
    | %     - SIGN_WHITE:  Modalità Default (Normale).
    | %     - SIGN_ORANGE: Modalità Sport (Prestazioni elevate/Attenzione).
    | %     - SIGN_GREEN:  Modalità Eco (Risparmio energetico).
    | %     - SIGN_OFF:    Stato di errore o non definito.
    | 
    |     switch decision.mode
    |         case ROVER_MODE.DEFAULT
    |             % Configurazione Standard: Colore Bianco.
    |             color = REAR_SIGN_TYPE.SIGN_WHITE;
    | 
    |         case ROVER_MODE.SPORT
    |             % Configurazione Performance: Colore Arancione.
    |             color = REAR_SIGN_TYPE.SIGN_ORANGE;
    | 
    |         case ROVER_MODE.ECO
    |             % Configurazione Risparmio: Colore Verde.
    |             color = REAR_SIGN_TYPE.SIGN_GREEN;
    | 
    |         otherwise
    |             % Fallback di Sicurezza (Fail-Safe).
    |             % Se la modalità non è riconosciuta o è corrotta, il pannello 
    |             % viene spento per evitare segnalazioni ambigue.
    |             color = REAR_SIGN_TYPE.SIGN_OFF;
    |     end
    | end
  function y = Lights_B_Pressed:
    | function y = Lights_B_Pressed
    | % Rileva il Fronte di Salita del pulsante luci.
    | %
    | % Descrizione:
    | %   Monitora il pulsante dello stick destro del controller.
    | %   Restituisce true solo nell'istante della pressione.
    | %
    | % Output:
    | %   - y: Boolean (true = comando cambio luci rilevato).
    | 
    |     persistent prev_r_stick_button;
    |     
    |     % Inizializza memoria
    |     if isempty(prev_r_stick_button)
    |         prev_r_stick_button = false;
    |     end
    |     
    |     if ~STEP
    |         y = false;
    |         return;
    |     end
    |     
    |     % Acquisizione stato dal Global State
    |     current_r_stick_button = global_state.stateB2.r_stick_button;
    |     
    |     % Rilevamento Rising Edge
    |     y = (current_r_stick_button == true) && (prev_r_stick_button == false);
    |     
    |     % Aggiornamento memoria
    |     prev_r_stick_button = current_r_stick_button;
    |     
    | end
